simulink model "Tphase"  (R2017a)
settings: Solver=FixedStepDiscrete  StartTime=0.0  StopTime=0.125 - 5e-5  MaxStep=1e-4  RelTol=1e-3
libraries: powerlib x256, auto_lib x2
settings Model: Creator=ioanna  LastModifiedBy=ioanna

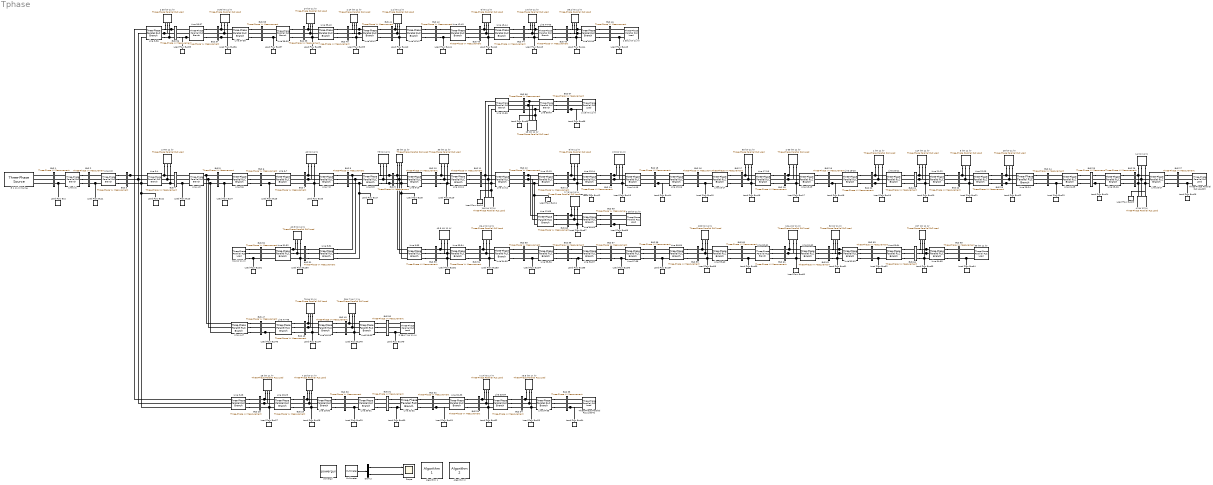
== system Tphase ==
  1 kW 11 kV : powerlib/Elements/Three-Phase Parallel RLC Load  LConnTagsString=A|B|C  Configuration=Y (grounded)  NominalVoltage=11e3  Vabc=[1e3 1e3 1e3]  Vabcp=[1e3 1e3 1e3]  NominalFrequency=50  UnbalancedPower=off  ActivePower=1e3  InductivePower=100  CapacitivePower=0  Pabc=[10e3 9e3 11e3]  QLabc=[100 90 110]  QCabc=[100 90 110]  Pabcp=[10e3 9e3 11e3]  QLabcp=[100 90 110]  QCabcp=[100 90 110]  Measurements=None  LoadType=constant Z
  1.2 kW 11 kV : powerlib/Elements/Three-Phase Parallel RLC Load  LConnTagsString=A|B|C  Configuration=Y (grounded)  NominalVoltage=11e3  Vabc=[1e3 1e3 1e3]  Vabcp=[1e3 1e3 1e3]  NominalFrequency=50  UnbalancedPower=off  ActivePower=1.2e3  InductivePower=100  CapacitivePower=0  Pabc=[10e3 9e3 11e3]  QLabc=[100 90 110]  QCabc=[100 90 110]  Pabcp=[10e3 9e3 11e3]  QLabcp=[100 90 110]  QCabcp=[100 90 110]  Measurements=None  LoadType=constant Z
  100 kW 11 kV : powerlib/Elements/Three-Phase Parallel RLC Load  LConnTagsString=A|B|C  Configuration=Y (grounded)  NominalVoltage=11e3  Vabc=[1e3 1e3 1e3]  Vabcp=[1e3 1e3 1e3]  NominalFrequency=50  UnbalancedPower=off  ActivePower=100e3  InductivePower=100  CapacitivePower=100  Pabc=[10e3 9e3 11e3]  QLabc=[100 90 110]  QCabc=[100 90 110]  Pabcp=[10e3 9e3 11e3]  QLabcp=[100 90 110]  QCabcp=[100 90 110]  Measurements=None  LoadType=constant Z
  114 kW 11 kV : powerlib/Elements/Three-Phase Parallel RLC Load  LConnTagsString=A|B|C  Configuration=Y (grounded)  NominalVoltage=11e3  Vabc=[1e3 1e3 1e3]  Vabcp=[1e3 1e3 1e3]  NominalFrequency=50  UnbalancedPower=off  ActivePower=114e3  InductivePower=100  CapacitivePower=0  Pabc=[10e3 9e3 11e3]  QLabc=[100 90 110]  QCabc=[100 90 110]  Pabcp=[10e3 9e3 11e3]  QLabcp=[100 90 110]  QCabcp=[100 90 110]  Measurements=None  LoadType=constant Z
  1244 kW 11 kV : powerlib/Elements/Three-Phase Parallel RLC Load  LConnTagsString=A|B|C  Configuration=Y (grounded)  NominalVoltage=11e3  Vabc=[1e3 1e3 1e3]  Vabcp=[1e3 1e3 1e3]  NominalFrequency=50  UnbalancedPower=off  ActivePower=1244e3  InductivePower=100  CapacitivePower=100  Pabc=[10e3 9e3 11e3]  QLabc=[100 90 110]  QCabc=[100 90 110]  Pabcp=[10e3 9e3 11e3]  QLabcp=[100 90 110]  QCabcp=[100 90 110]  Measurements=None  LoadType=constant Z
  14 kW 11 kV : powerlib/Elements/Three-Phase Parallel RLC Load  LConnTagsString=A|B|C  Configuration=Y (grounded)  NominalVoltage=11e3  Vabc=[1e3 1e3 1e3]  Vabcp=[1e3 1e3 1e3]  NominalFrequency=50  UnbalancedPower=off  ActivePower=14e3  InductivePower=100  CapacitivePower=0  Pabc=[10e3 9e3 11e3]  QLabc=[100 90 110]  QCabc=[100 90 110]  Pabcp=[10e3 9e3 11e3]  QLabcp=[100 90 110]  QCabcp=[100 90 110]  Measurements=None  LoadType=constant Z
  145 kW 11 kV : powerlib/Elements/Three-Phase Parallel RLC Load  LConnTagsString=A|B|C  Configuration=Y (grounded)  NominalVoltage=11e3  Vabc=[1e3 1e3 1e3]  Vabcp=[1e3 1e3 1e3]  NominalFrequency=50  UnbalancedPower=off  ActivePower=145e3  InductivePower=100  CapacitivePower=0  Pabc=[10e3 9e3 11e3]  QLabc=[100 90 110]  QCabc=[100 90 110]  Pabcp=[10e3 9e3 11e3]  QLabcp=[100 90 110]  QCabcp=[100 90 110]  Measurements=None  LoadType=constant Z
  18 kW 11 kV : powerlib/Elements/Three-Phase Parallel RLC Load  LConnTagsString=A|B|C  Configuration=Y (grounded)  NominalVoltage=11e3  Vabc=[1e3 1e3 1e3]  Vabcp=[1e3 1e3 1e3]  NominalFrequency=50  UnbalancedPower=off  ActivePower=18e3  InductivePower=100  CapacitivePower=0  Pabc=[10e3 9e3 11e3]  QLabc=[100 90 110]  QCabc=[100 90 110]  Pabcp=[10e3 9e3 11e3]  QLabcp=[100 90 110]  QCabcp=[100 90 110]  Measurements=None  LoadType=constant Z
  19.5 kW 11 kV : powerlib/Elements/Three-Phase Parallel RLC Load  LConnTagsString=A|B|C  Configuration=Y (grounded)  NominalVoltage=11e3  Vabc=[1e3 1e3 1e3]  Vabcp=[1e3 1e3 1e3]  NominalFrequency=50  UnbalancedPower=off  ActivePower=19.5e3  InductivePower=100  CapacitivePower=100  Pabc=[10e3 9e3 11e3]  QLabc=[100 90 110]  QCabc=[100 90 110]  Pabcp=[10e3 9e3 11e3]  QLabcp=[100 90 110]  QCabcp=[100 90 110]  Measurements=None  LoadType=constant Z
  2 14 kW 11 kV : powerlib/Elements/Three-Phase Parallel RLC Load  LConnTagsString=A|B|C  Configuration=Y (grounded)  NominalVoltage=11e3  Vabc=[1e3 1e3 1e3]  Vabcp=[1e3 1e3 1e3]  NominalFrequency=50  UnbalancedPower=off  ActivePower=14e3  InductivePower=100  CapacitivePower=100  Pabc=[10e3 9e3 11e3]  QLabc=[100 90 110]  QCabc=[100 90 110]  Pabcp=[10e3 9e3 11e3]  QLabcp=[100 90 110]  QCabcp=[100 90 110]  Measurements=None  LoadType=constant Z
  2 18 kW 11 kV : powerlib/Elements/Three-Phase Parallel RLC Load  LConnTagsString=A|B|C  Configuration=Y (grounded)  NominalVoltage=11e3  Vabc=[1e3 1e3 1e3]  Vabcp=[1e3 1e3 1e3]  NominalFrequency=50  UnbalancedPower=off  ActivePower=18e3  InductivePower=100  CapacitivePower=100  Pabc=[10e3 9e3 11e3]  QLabc=[100 90 110]  QCabc=[100 90 110]  Pabcp=[10e3 9e3 11e3]  QLabcp=[100 90 110]  QCabcp=[100 90 110]  Measurements=None  LoadType=constant Z
  2 24 kW 11 kV : powerlib/Elements/Three-Phase Parallel RLC Load  LConnTagsString=A|B|C  Configuration=Y (grounded)  NominalVoltage=11e3  Vabc=[1e3 1e3 1e3]  Vabcp=[1e3 1e3 1e3]  NominalFrequency=50  UnbalancedPower=off  ActivePower=24e3  InductivePower=100  CapacitivePower=0  Pabc=[10e3 9e3 11e3]  QLabc=[100 90 110]  QCabc=[100 90 110]  Pabcp=[10e3 9e3 11e3]  QLabcp=[100 90 110]  QCabcp=[100 90 110]  Measurements=None  LoadType=constant Z
  2 26 kW 11 kV : powerlib/Elements/Three-Phase Parallel RLC Load  LConnTagsString=A|B|C  Configuration=Y (grounded)  NominalVoltage=11e3  Vabc=[1e3 1e3 1e3]  Vabcp=[1e3 1e3 1e3]  NominalFrequency=50  UnbalancedPower=off  ActivePower=26e3  InductivePower=100  CapacitivePower=100  Pabc=[10e3 9e3 11e3]  QLabc=[100 90 110]  QCabc=[100 90 110]  Pabcp=[10e3 9e3 11e3]  QLabcp=[100 90 110]  QCabcp=[100 90 110]  Measurements=None  LoadType=constant Z
  2 28 kW 11 kV : powerlib/Elements/Three-Phase Parallel RLC Load  LConnTagsString=A|B|C  Configuration=Y (grounded)  NominalVoltage=11e3  Vabc=[1e3 1e3 1e3]  Vabcp=[1e3 1e3 1e3]  NominalFrequency=50  UnbalancedPower=off  ActivePower=28e3  InductivePower=100  CapacitivePower=0  Pabc=[10e3 9e3 11e3]  QLabc=[100 90 110]  QCabc=[100 90 110]  Pabcp=[10e3 9e3 11e3]  QLabcp=[100 90 110]  QCabcp=[100 90 110]  Measurements=None  LoadType=constant Z
  2 30 kW 11 kV : powerlib/Elements/Three-Phase Parallel RLC Load  LConnTagsString=A|B|C  Configuration=Y (grounded)  NominalVoltage=11e3  Vabc=[1e3 1e3 1e3]  Vabcp=[1e3 1e3 1e3]  NominalFrequency=50  UnbalancedPower=off  ActivePower=30e3  InductivePower=100  CapacitivePower=0  Pabc=[10e3 9e3 11e3]  QLabc=[100 90 110]  QCabc=[100 90 110]  Pabcp=[10e3 9e3 11e3]  QLabcp=[100 90 110]  QCabcp=[100 90 110]  Measurements=None  LoadType=constant Z
  2 384.7 kW 11 kV : powerlib/Elements/Three-Phase Parallel RLC Load  LConnTagsString=A|B|C  Configuration=Y (grounded)  NominalVoltage=11e3  Vabc=[1e3 1e3 1e3]  Vabcp=[1e3 1e3 1e3]  NominalFrequency=50  UnbalancedPower=off  ActivePower=384.7e3  InductivePower=100  CapacitivePower=0  Pabc=[10e3 9e3 11e3]  QLabc=[100 90 110]  QCabc=[100 90 110]  Pabcp=[10e3 9e3 11e3]  QLabcp=[100 90 110]  QCabcp=[100 90 110]  Measurements=None  LoadType=constant Z
  2 39.2 kW 11 kV : powerlib/Elements/Three-Phase Parallel RLC Load  LConnTagsString=A|B|C  Configuration=Y (grounded)  NominalVoltage=11e3  Vabc=[1e3 1e3 1e3]  Vabcp=[1e3 1e3 1e3]  NominalFrequency=50  UnbalancedPower=off  ActivePower=39.2e3  InductivePower=100  CapacitivePower=100  Pabc=[10e3 9e3 11e3]  QLabc=[100 90 110]  QCabc=[100 90 110]  Pabcp=[10e3 9e3 11e3]  QLabcp=[100 90 110]  QCabcp=[100 90 110]  Measurements=None  LoadType=constant Z
  2 6 kW 11 kV : powerlib/Elements/Three-Phase Parallel RLC Load  LConnTagsString=A|B|C  Configuration=Y (grounded)  NominalVoltage=11e3  Vabc=[1e3 1e3 1e3]  Vabcp=[1e3 1e3 1e3]  NominalFrequency=50  UnbalancedPower=off  ActivePower=6e3  InductivePower=100  CapacitivePower=100  Pabc=[10e3 9e3 11e3]  QLabc=[100 90 110]  QCabc=[100 90 110]  Pabcp=[10e3 9e3 11e3]  QLabcp=[100 90 110]  QCabcp=[100 90 110]  Measurements=None  LoadType=constant Z
  2 60 kW 11 kV : powerlib/Elements/Three-Phase Parallel RLC Load  LConnTagsString=A|B|C  Configuration=Y (grounded)  NominalVoltage=11e3  Vabc=[1e3 1e3 1e3]  Vabcp=[1e3 1e3 1e3]  NominalFrequency=50  UnbalancedPower=off  ActivePower=60e3  InductivePower=100  CapacitivePower=0  Pabc=[10e3 9e3 11e3]  QLabc=[100 90 110]  QCabc=[100 90 110]  Pabcp=[10e3 9e3 11e3]  QLabcp=[100 90 110]  QCabcp=[100 90 110]  Measurements=None  LoadType=constant Z
  2 8 kW 11 kV : powerlib/Elements/Three-Phase Parallel RLC Load  LConnTagsString=A|B|C  Configuration=Y (grounded)  NominalVoltage=11e3  Vabc=[1e3 1e3 1e3]  Vabcp=[1e3 1e3 1e3]  NominalFrequency=50  UnbalancedPower=off  ActivePower=8e3  InductivePower=100  CapacitivePower=0  Pabc=[10e3 9e3 11e3]  QLabc=[100 90 110]  QCabc=[100 90 110]  Pabcp=[10e3 9e3 11e3]  QLabcp=[100 90 110]  QCabcp=[100 90 110]  Measurements=None  LoadType=constant Z
  2 MW 11 kV : powerlib/Elements/Three-Phase Parallel RLC Load  LConnTagsString=A|B|C  Configuration=Y (grounded)  NominalVoltage=11e3  Vabc=[1e3 1e3 1e3]  Vabcp=[1e3 1e3 1e3]  NominalFrequency=50  UnbalancedPower=off  ActivePower=2e6  InductivePower=100  CapacitivePower=100  Pabc=[10e3 9e3 11e3]  QLabc=[100 90 110]  QCabc=[100 90 110]  Pabcp=[10e3 9e3 11e3]  QLabcp=[100 90 110]  QCabcp=[100 90 110]  Measurements=Branch voltages and currents  LoadType=constant Z
  227 kW 11 kV : powerlib/Elements/Three-Phase Parallel RLC Load  LConnTagsString=A|B|C  Configuration=Y (grounded)  NominalVoltage=11e3  Vabc=[1e3 1e3 1e3]  Vabcp=[1e3 1e3 1e3]  NominalFrequency=50  UnbalancedPower=off  ActivePower=227e3  InductivePower=100  CapacitivePower=100  Pabc=[10e3 9e3 11e3]  QLabc=[100 90 110]  QCabc=[100 90 110]  Pabcp=[10e3 9e3 11e3]  QLabcp=[100 90 110]  QCabcp=[100 90 110]  Measurements=None  LoadType=constant Z
  24 kW 11 kV : powerlib/Elements/Three-Phase Parallel RLC Load  LConnTagsString=A|B|C  Configuration=Y (grounded)  NominalVoltage=11e3  Vabc=[1e3 1e3 1e3]  Vabcp=[1e3 1e3 1e3]  NominalFrequency=50  UnbalancedPower=off  ActivePower=24e3  InductivePower=100  CapacitivePower=0  Pabc=[10e3 9e3 11e3]  QLabc=[100 90 110]  QCabc=[100 90 110]  Pabcp=[10e3 9e3 11e3]  QLabcp=[100 90 110]  QCabcp=[100 90 110]  Measurements=None  LoadType=constant Z
  26 kW 11 kV : powerlib/Elements/Three-Phase Parallel RLC Load  LConnTagsString=A|B|C  Configuration=Y (grounded)  NominalVoltage=11e3  Vabc=[1e3 1e3 1e3]  Vabcp=[1e3 1e3 1e3]  NominalFrequency=50  UnbalancedPower=off  ActivePower=26e3  InductivePower=100  CapacitivePower=100  Pabc=[10e3 9e3 11e3]  QLabc=[100 90 110]  QCabc=[100 90 110]  Pabcp=[10e3 9e3 11e3]  QLabcp=[100 90 110]  QCabcp=[100 90 110]  Measurements=None  LoadType=constant Z
  26.4 kW 11 kV : powerlib/Elements/Three-Phase Parallel RLC Load  LConnTagsString=A|B|C  Configuration=Y (grounded)  NominalVoltage=11e3  Vabc=[1e3 1e3 1e3]  Vabcp=[1e3 1e3 1e3]  NominalFrequency=50  UnbalancedPower=off  ActivePower=26.4e3  InductivePower=100  CapacitivePower=100  Pabc=[10e3 9e3 11e3]  QLabc=[100 90 110]  QCabc=[100 90 110]  Pabcp=[10e3 9e3 11e3]  QLabcp=[100 90 110]  QCabcp=[100 90 110]  Measurements=None  LoadType=constant Z
  28 kW 11 kV : powerlib/Elements/Three-Phase Parallel RLC Load  LConnTagsString=A|B|C  Configuration=Y (grounded)  NominalVoltage=11e3  Vabc=[1e3 1e3 1e3]  Vabcp=[1e3 1e3 1e3]  NominalFrequency=50  UnbalancedPower=off  ActivePower=28e3  InductivePower=100  CapacitivePower=0  Pabc=[10e3 9e3 11e3]  QLabc=[100 90 110]  QCabc=[100 90 110]  Pabcp=[10e3 9e3 11e3]  QLabcp=[100 90 110]  QCabcp=[100 90 110]  Measurements=None  LoadType=constant Z
  3 28 kW 11 kV : powerlib/Elements/Three-Phase Parallel RLC Load  LConnTagsString=A|B|C  Configuration=Y (grounded)  NominalVoltage=11e3  Vabc=[1e3 1e3 1e3]  Vabcp=[1e3 1e3 1e3]  NominalFrequency=50  UnbalancedPower=off  ActivePower=28e3  InductivePower=100  CapacitivePower=0  Pabc=[10e3 9e3 11e3]  QLabc=[100 90 110]  QCabc=[100 90 110]  Pabcp=[10e3 9e3 11e3]  QLabcp=[100 90 110]  QCabcp=[100 90 110]  Measurements=None  LoadType=constant Z
  3 30 kW 11 kV : powerlib/Elements/Three-Phase Parallel RLC Load  LConnTagsString=A|B|C  Configuration=Y (grounded)  NominalVoltage=11e3  Vabc=[1e3 1e3 1e3]  Vabcp=[1e3 1e3 1e3]  NominalFrequency=50  UnbalancedPower=off  ActivePower=30e3  InductivePower=100  CapacitivePower=0  Pabc=[10e3 9e3 11e3]  QLabc=[100 90 110]  QCabc=[100 90 110]  Pabcp=[10e3 9e3 11e3]  QLabcp=[100 90 110]  QCabcp=[100 90 110]  Measurements=None  LoadType=constant Z
  3.6 kW 11 kV : powerlib/Elements/Three-Phase Parallel RLC Load  LConnTagsString=A|B|C  Configuration=Y (grounded)  NominalVoltage=11e3  Vabc=[1e3 1e3 1e3]  Vabcp=[1e3 1e3 1e3]  NominalFrequency=50  UnbalancedPower=off  ActivePower=3.6e3  InductivePower=100  CapacitivePower=100  Pabc=[10e3 9e3 11e3]  QLabc=[100 90 110]  QCabc=[100 90 110]  Pabcp=[10e3 9e3 11e3]  QLabcp=[100 90 110]  QCabcp=[100 90 110]  Measurements=None  LoadType=constant Z
  30 kW 11 kV : powerlib/Elements/Three-Phase Parallel RLC Load  LConnTagsString=A|B|C  Configuration=Y (grounded)  NominalVoltage=11e3  Vabc=[1e3 1e3 1e3]  Vabcp=[1e3 1e3 1e3]  NominalFrequency=50  UnbalancedPower=off  ActivePower=30e3  InductivePower=100  CapacitivePower=1000  Pabc=[10e3 9e3 11e3]  QLabc=[100 90 110]  QCabc=[100 90 110]  Pabcp=[10e3 9e3 11e3]  QLabcp=[100 90 110]  QCabcp=[100 90 110]  Measurements=None  LoadType=constant Z
  30 kW 11 kV : powerlib/Elements/Three-Phase Parallel RLC Load  LConnTagsString=A|B|C  Configuration=Y (grounded)  NominalVoltage=11e3  Vabc=[1e3 1e3 1e3]  Vabcp=[1e3 1e3 1e3]  NominalFrequency=50  UnbalancedPower=off  ActivePower=30e3  InductivePower=100  CapacitivePower=0  Pabc=[10e3 9e3 11e3]  QLabc=[100 90 110]  QCabc=[100 90 110]  Pabcp=[10e3 9e3 11e3]  QLabcp=[100 90 110]  QCabcp=[100 90 110]  Measurements=None  LoadType=constant Z
  32 kW 11 kV : powerlib/Elements/Three-Phase Parallel RLC Load  LConnTagsString=A|B|C  Configuration=Y (grounded)  NominalVoltage=11e3  Vabc=[1e3 1e3 1e3]  Vabcp=[1e3 1e3 1e3]  NominalFrequency=50  UnbalancedPower=off  ActivePower=32e3  InductivePower=100  CapacitivePower=100  Pabc=[10e3 9e3 11e3]  QLabc=[100 90 110]  QCabc=[100 90 110]  Pabcp=[10e3 9e3 11e3]  QLabcp=[100 90 110]  QCabcp=[100 90 110]  Measurements=None  LoadType=constant Z
  384.7 kW 11 kV : powerlib/Elements/Three-Phase Parallel RLC Load  LConnTagsString=A|B|C  Configuration=Y (grounded)  NominalVoltage=11e3  Vabc=[1e3 1e3 1e3]  Vabcp=[1e3 1e3 1e3]  NominalFrequency=50  UnbalancedPower=off  ActivePower=384.7e3  InductivePower=100  CapacitivePower=0  Pabc=[10e3 9e3 11e3]  QLabc=[100 90 110]  QCabc=[100 90 110]  Pabcp=[10e3 9e3 11e3]  QLabcp=[100 90 110]  QCabcp=[100 90 110]  Measurements=None  LoadType=constant Z
  39.2 kW 11 kV : powerlib/Elements/Three-Phase Parallel RLC Load  LConnTagsString=A|B|C  Configuration=Y (grounded)  NominalVoltage=11e3  Vabc=[1e3 1e3 1e3]  Vabcp=[1e3 1e3 1e3]  NominalFrequency=50  UnbalancedPower=off  ActivePower=39.2e3  InductivePower=100  CapacitivePower=100  Pabc=[10e3 9e3 11e3]  QLabc=[100 90 110]  QCabc=[100 90 110]  Pabcp=[10e3 9e3 11e3]  QLabcp=[100 90 110]  QCabcp=[100 90 110]  Measurements=None  LoadType=constant Z
  4 MW 11 kV : powerlib/Elements/Three-Phase Parallel RLC Load  LConnTagsString=A|B|C  Configuration=Y (grounded)  NominalVoltage=11e3  Vabc=[1e3 1e3 1e3]  Vabcp=[1e3 1e3 1e3]  NominalFrequency=50  UnbalancedPower=off  ActivePower=4e6  InductivePower=100  CapacitivePower=100  Pabc=[10e3 9e3 11e3]  QLabc=[100 90 110]  QCabc=[100 90 110]  Pabcp=[10e3 9e3 11e3]  QLabcp=[100 90 110]  QCabcp=[100 90 110]  Measurements=None  LoadType=constant Z
  40 kW 11 kV : powerlib/Elements/Three-Phase Parallel RLC Load  LConnTagsString=A|B|C  Configuration=Y (grounded)  NominalVoltage=11e3  Vabc=[1e3 1e3 1e3]  Vabcp=[1e3 1e3 1e3]  NominalFrequency=50  UnbalancedPower=off  ActivePower=40e3  InductivePower=0  CapacitivePower=100  Pabc=[10e3 9e3 11e3]  QLabc=[100 90 110]  QCabc=[100 90 110]  Pabcp=[10e3 9e3 11e3]  QLabcp=[100 90 110]  QCabcp=[100 90 110]  Measurements=None  LoadType=constant Z
  40.5 kW 11 kV : powerlib/Elements/Three-Phase Parallel RLC Load  LConnTagsString=A|B|C  Configuration=Y (grounded)  NominalVoltage=11e3  Vabc=[1e3 1e3 1e3]  Vabcp=[1e3 1e3 1e3]  NominalFrequency=50  UnbalancedPower=off  ActivePower=40.5e3  InductivePower=100  CapacitivePower=0  Pabc=[10e3 9e3 11e3]  QLabc=[100 90 110]  QCabc=[100 90 110]  Pabcp=[10e3 9e3 11e3]  QLabcp=[100 90 110]  QCabcp=[100 90 110]  Measurements=None  LoadType=constant Z
  43.5 kW 11 kV : powerlib/Elements/Three-Phase Parallel RLC Load  LConnTagsString=A|B|C  Configuration=Y (grounded)  NominalVoltage=11e3  Vabc=[1e3 1e3 1e3]  Vabcp=[1e3 1e3 1e3]  NominalFrequency=50  UnbalancedPower=off  ActivePower=43.5e3  InductivePower=100  CapacitivePower=100  Pabc=[10e3 9e3 11e3]  QLabc=[100 90 110]  QCabc=[100 90 110]  Pabcp=[10e3 9e3 11e3]  QLabcp=[100 90 110]  QCabcp=[100 90 110]  Measurements=None  LoadType=constant Z
  5 kW 11 kV : powerlib/Elements/Three-Phase Parallel RLC Load  LConnTagsString=A|B|C  Configuration=Y (grounded)  NominalVoltage=11e3  Vabc=[1e3 1e3 1e3]  Vabcp=[1e3 1e3 1e3]  NominalFrequency=50  UnbalancedPower=off  ActivePower=5e3  InductivePower=100  CapacitivePower=0  Pabc=[10e3 9e3 11e3]  QLabc=[100 90 110]  QCabc=[100 90 110]  Pabcp=[10e3 9e3 11e3]  QLabcp=[100 90 110]  QCabcp=[100 90 110]  Measurements=None  LoadType=constant Z
  59 kW 11 kV : powerlib/Elements/Three-Phase Parallel RLC Load  LConnTagsString=A|B|C  Configuration=Y (grounded)  NominalVoltage=11e3  Vabc=[1e3 1e3 1e3]  Vabcp=[1e3 1e3 1e3]  NominalFrequency=50  UnbalancedPower=off  ActivePower=59e3  InductivePower=100  CapacitivePower=100  Pabc=[10e3 9e3 11e3]  QLabc=[100 90 110]  QCabc=[100 90 110]  Pabcp=[10e3 9e3 11e3]  QLabcp=[100 90 110]  QCabcp=[100 90 110]  Measurements=None  LoadType=constant Z
  6 kW 11 kV : powerlib/Elements/Three-Phase Parallel RLC Load  LConnTagsString=A|B|C  Configuration=Y (grounded)  NominalVoltage=11e3  Vabc=[1e3 1e3 1e3]  Vabcp=[1e3 1e3 1e3]  NominalFrequency=50  UnbalancedPower=off  ActivePower=6e3  InductivePower=100  CapacitivePower=100  Pabc=[10e3 9e3 11e3]  QLabc=[100 90 110]  QCabc=[100 90 110]  Pabcp=[10e3 9e3 11e3]  QLabcp=[100 90 110]  QCabcp=[100 90 110]  Measurements=None  LoadType=constant Z
  60 kW 11 kV : powerlib/Elements/Three-Phase Parallel RLC Load  LConnTagsString=A|B|C  Configuration=Y (grounded)  NominalVoltage=11e3  Vabc=[1e3 1e3 1e3]  Vabcp=[1e3 1e3 1e3]  NominalFrequency=50  UnbalancedPower=off  ActivePower=60e3  InductivePower=100  CapacitivePower=0  Pabc=[10e3 9e3 11e3]  QLabc=[100 90 110]  QCabc=[100 90 110]  Pabcp=[10e3 9e3 11e3]  QLabcp=[100 90 110]  QCabcp=[100 90 110]  Measurements=None  LoadType=constant Z
  75 kW 11 kV : powerlib/Elements/Three-Phase Parallel RLC Load  LConnTagsString=A|B|C  Configuration=Y (grounded)  NominalVoltage=11e3  Vabc=[1e3 1e3 1e3]  Vabcp=[1e3 1e3 1e3]  NominalFrequency=50  UnbalancedPower=off  ActivePower=75e3  InductivePower=100  CapacitivePower=0  Pabc=[10e3 9e3 11e3]  QLabc=[100 90 110]  QCabc=[100 90 110]  Pabcp=[10e3 9e3 11e3]  QLabcp=[100 90 110]  QCabcp=[100 90 110]  Measurements=None  LoadType=constant Z
  79 kW 11 kV : powerlib/Elements/Three-Phase Parallel RLC Load  LConnTagsString=A|B|C  Configuration=Y (grounded)  NominalVoltage=11e3  Vabc=[1e3 1e3 1e3]  Vabcp=[1e3 1e3 1e3]  NominalFrequency=50  UnbalancedPower=off  ActivePower=79e3  InductivePower=100  CapacitivePower=0  Pabc=[10e3 9e3 11e3]  QLabc=[100 90 110]  QCabc=[100 90 110]  Pabcp=[10e3 9e3 11e3]  QLabcp=[100 90 110]  QCabcp=[100 90 110]  Measurements=None  LoadType=constant Z
  8 kW 11 kV : powerlib/Elements/Three-Phase Parallel RLC Load  LConnTagsString=A|B|C  Configuration=Y (grounded)  NominalVoltage=11e3  Vabc=[1e3 1e3 1e3]  Vabcp=[1e3 1e3 1e3]  NominalFrequency=50  UnbalancedPower=off  ActivePower=8e3  InductivePower=100  CapacitivePower=0  Pabc=[10e3 9e3 11e3]  QLabc=[100 90 110]  QCabc=[100 90 110]  Pabcp=[10e3 9e3 11e3]  QLabcp=[100 90 110]  QCabcp=[100 90 110]  Measurements=None  LoadType=constant Z
  Algorithm 1 : auto_lib/Algorithm 1  SystemSampleTime=-1
  Algorithm 2 : auto_lib/Algorithm 2  SystemSampleTime=-1
  BUS {1..69} (69 alike) : powerlib/Measurements/Three-Phase V-I Measurement  VoltageMeasurement=no  SetLabelV=off  LabelV=Vabc  Vpu=off  VpuLL=off  CurrentMeasurement=no  SetLabelI=off  LabelI=Iabc  Ipu=off  Pbase=100e6  Vbase=500e3  OutputType=Complex  PhasorSimulation=off  PSBequivalent=0
  Demux : Demux  Outputs=2
  G 1 11 kV Swing : powerlib/Electrical Sources/Three-Phase Source  InternalConnection=Yg  VoltagePhases=off  Voltage=11e3  PhaseAngle=0  Voltage_phases=[25e3 25e3 25e3]/sqrt(3)  PhaseAngles_phases=[0 -120 +120]  Frequency=50  NonIdealSource=on  SpecifyImpedance=off  Resistance=0.8929  Inductance=16.58e-3  ShortCircuitLevel=100e6  BaseVoltage=25e3  XRratio=7  BusType=swing  Pref=10e3  Qref=0  Prefabc=[10e3, 10e3, 10e3]  Qrefabc=[0, 0, 0]  Qmin=-inf  Qmax=inf
  Line 1-2 : powerlib/Elements/Three-Phase Parallel RLC Branch  LConnTagsString=A|B|C  RConnTagsString=A|B|C  BranchType=RL  Resistance=0.0005  Inductance=0.0012  Capacitance=1e-6  Measurements=None
      settings: SourceProductName=Simscape Power Systems  SourceProductBaseCode=PS
  Line 10-11 : powerlib/Elements/Three-Phase Parallel RLC Branch  LConnTagsString=A|B|C  RConnTagsString=A|B|C  BranchType=RL  Resistance=0.1872  Inductance=0.0619  Capacitance=1e-6  Measurements=None
      settings: SourceProductName=Simscape Power Systems  SourceProductBaseCode=PS
  Line 11-12 : powerlib/Elements/Three-Phase Parallel RLC Branch  LConnTagsString=A|B|C  RConnTagsString=A|B|C  BranchType=RL  Resistance=0.7114  Inductance=0.2351  Capacitance=1e-6  Measurements=None
      settings: SourceProductName=Simscape Power Systems  SourceProductBaseCode=PS
  Line 11-66 : powerlib/Elements/Three-Phase Parallel RLC Branch  LConnTagsString=A|B|C  RConnTagsString=A|B|C  BranchType=RL  Resistance=0.2012  Inductance=0.0611  Capacitance=1e-6  Measurements=None
      settings: SourceProductName=Simscape Power Systems  SourceProductBaseCode=PS
  Line 12-13 : powerlib/Elements/Three-Phase Parallel RLC Branch  LConnTagsString=A|B|C  RConnTagsString=A|B|C  BranchType=RL  Resistance=1.03  Inductance=0.34  Capacitance=1e-6  Measurements=None
      settings: SourceProductName=Simscape Power Systems  SourceProductBaseCode=PS
  Line 12-68 : powerlib/Elements/Three-Phase Parallel RLC Branch  LConnTagsString=A|B|C  RConnTagsString=A|B|C  BranchType=RL  Resistance=0.7394  Inductance=0.2444  Capacitance=1e-6  Measurements=None
      settings: SourceProductName=Simscape Power Systems  SourceProductBaseCode=PS
  Line 13-14 : powerlib/Elements/Three-Phase Parallel RLC Branch  LConnTagsString=A|B|C  RConnTagsString=A|B|C  BranchType=RL  Resistance=1.044  Inductance=0.345  Capacitance=1e-6  Measurements=None
      settings: SourceProductName=Simscape Power Systems  SourceProductBaseCode=PS
  Line 14-15 : powerlib/Elements/Three-Phase Parallel RLC Branch  LConnTagsString=A|B|C  RConnTagsString=A|B|C  BranchType=RL  Resistance=1.058  Inductance=0.3496  Capacitance=1e-6  Measurements=None
      settings: SourceProductName=Simscape Power Systems  SourceProductBaseCode=PS
  Line 15-16 : powerlib/Elements/Three-Phase Parallel RLC Branch  LConnTagsString=A|B|C  RConnTagsString=A|B|C  BranchType=RL  Resistance=0.1966  Inductance=0.065  Capacitance=1e-6  Measurements=None
      settings: SourceProductName=Simscape Power Systems  SourceProductBaseCode=PS
  Line 16-17 : powerlib/Elements/Three-Phase Parallel RLC Branch  LConnTagsString=A|B|C  RConnTagsString=A|B|C  BranchType=RL  Resistance=0.3744  Inductance=0.1238  Capacitance=1e-6  Measurements=None
      settings: SourceProductName=Simscape Power Systems  SourceProductBaseCode=PS
  Line 17-18 : powerlib/Elements/Three-Phase Parallel RLC Branch  LConnTagsString=A|B|C  RConnTagsString=A|B|C  BranchType=RL  Resistance=0.0047  Inductance=0.0016  Capacitance=1e-6  Measurements=None
      settings: SourceProductName=Simscape Power Systems  SourceProductBaseCode=PS
  Line 18-19 : powerlib/Elements/Three-Phase Parallel RLC Branch  LConnTagsString=A|B|C  RConnTagsString=A|B|C  BranchType=RL  Resistance=0.3276  Inductance=0.1083  Capacitance=1e-6  Measurements=None
      settings: SourceProductName=Simscape Power Systems  SourceProductBaseCode=PS
  Line 19-20 : powerlib/Elements/Three-Phase Parallel RLC Branch  LConnTagsString=A|B|C  RConnTagsString=A|B|C  BranchType=RL  Resistance=0.2106  Inductance=0.069  Capacitance=1e-6  Measurements=None
      settings: SourceProductName=Simscape Power Systems  SourceProductBaseCode=PS
  Line 2-3 : powerlib/Elements/Three-Phase Parallel RLC Branch  LConnTagsString=A|B|C  RConnTagsString=A|B|C  BranchType=RL  Resistance=0.0005  Inductance=0.0012  Capacitance=1e-6  Measurements=None
      settings: SourceProductName=Simscape Power Systems  SourceProductBaseCode=PS
  Line 20-21 : powerlib/Elements/Three-Phase Parallel RLC Branch  LConnTagsString=A|B|C  RConnTagsString=A|B|C  BranchType=RL  Resistance=0.3416  Inductance=0.1129  Capacitance=1e-6  Measurements=None
      settings: SourceProductName=Simscape Power Systems  SourceProductBaseCode=PS
  Line 21-22 : powerlib/Elements/Three-Phase Parallel RLC Branch  LConnTagsString=A|B|C  RConnTagsString=A|B|C  BranchType=RL  Resistance=0.014  Inductance=0.0046  Capacitance=1e-6  Measurements=None
      settings: SourceProductName=Simscape Power Systems  SourceProductBaseCode=PS
  Line 22-23 : powerlib/Elements/Three-Phase Parallel RLC Branch  LConnTagsString=A|B|C  RConnTagsString=A|B|C  BranchType=RL  Resistance=0.1591  Inductance=0.0526  Capacitance=1e-6  Measurements=None
      settings: SourceProductName=Simscape Power Systems  SourceProductBaseCode=PS
  Line 23-24 : powerlib/Elements/Three-Phase Parallel RLC Branch  LConnTagsString=A|B|C  RConnTagsString=A|B|C  BranchType=RL  Resistance=0.3469  Inductance=0.1145  Capacitance=1e-6  Measurements=None
      settings: SourceProductName=Simscape Power Systems  SourceProductBaseCode=PS
  Line 24-25 : powerlib/Elements/Three-Phase Parallel RLC Branch  LConnTagsString=A|B|C  RConnTagsString=A|B|C  BranchType=RL  Resistance=0.7488  Inductance=0.2475  Capacitance=1e-6  Measurements=None
      settings: SourceProductName=Simscape Power Systems  SourceProductBaseCode=PS
  Line 25-26 : powerlib/Elements/Three-Phase Parallel RLC Branch  LConnTagsString=A|B|C  RConnTagsString=A|B|C  BranchType=RL  Resistance=0.3089  Inductance=0.1021  Capacitance=1e-6  Measurements=None
      settings: SourceProductName=Simscape Power Systems  SourceProductBaseCode=PS
  Line 26-27 : powerlib/Elements/Three-Phase Parallel RLC Branch  LConnTagsString=A|B|C  RConnTagsString=A|B|C  BranchType=RL  Resistance=0.1732  Inductance=0.0572  Capacitance=1e-6  Measurements=None
      settings: SourceProductName=Simscape Power Systems  SourceProductBaseCode=PS
  Line 28-29 : powerlib/Elements/Three-Phase Parallel RLC Branch  LConnTagsString=A|B|C  RConnTagsString=A|B|C  BranchType=RL  Resistance=0.064  Inductance=0.1565  Capacitance=1e-6  Measurements=None
      settings: SourceProductName=Simscape Power Systems  SourceProductBaseCode=PS
  Line 29-30 : powerlib/Elements/Three-Phase Parallel RLC Branch  LConnTagsString=A|B|C  RConnTagsString=A|B|C  BranchType=RL  Resistance=0.3978  Inductance=0.1315  Capacitance=1e-6  Measurements=None
      settings: SourceProductName=Simscape Power Systems  SourceProductBaseCode=PS
  Line 3-28 : powerlib/Elements/Three-Phase Parallel RLC Branch  LConnTagsString=A|B|C  RConnTagsString=A|B|C  BranchType=RL  Resistance=0.0005  Inductance=0.0036  Capacitance=1e-6  Measurements=None
      settings: SourceProductName=Simscape Power Systems  SourceProductBaseCode=PS
  Line 3-36 : powerlib/Elements/Three-Phase Parallel RLC Branch  LConnTagsString=A|B|C  RConnTagsString=A|B|C  BranchType=RL  Resistance=0.0005  Inductance=0.0036  Capacitance=1e-6  Measurements=None
      settings: SourceProductName=Simscape Power Systems  SourceProductBaseCode=PS
  Line 3-4 : powerlib/Elements/Three-Phase Parallel RLC Branch  LConnTagsString=A|B|C  RConnTagsString=A|B|C  BranchType=RL  Resistance=0.0005  Inductance=0.0036  Capacitance=1e-6  Measurements=None
      settings: SourceProductName=Simscape Power Systems  SourceProductBaseCode=PS
  Line 30-31 : powerlib/Elements/Three-Phase Parallel RLC Branch  LConnTagsString=A|B|C  RConnTagsString=A|B|C  BranchType=RL  Resistance=0.0702  Inductance=0.0232  Capacitance=1e-6  Measurements=None
      settings: SourceProductName=Simscape Power Systems  SourceProductBaseCode=PS
  Line 31-32 : powerlib/Elements/Three-Phase Parallel RLC Branch  LConnTagsString=A|B|C  RConnTagsString=A|B|C  BranchType=RL  Resistance=0.351  Inductance=0.116  Capacitance=1e-6  Measurements=None
      settings: SourceProductName=Simscape Power Systems  SourceProductBaseCode=PS
  Line 32-33 : powerlib/Elements/Three-Phase Parallel RLC Branch  LConnTagsString=A|B|C  RConnTagsString=A|B|C  BranchType=RL  Resistance=0.839  Inductance=0.2816  Capacitance=1e-6  Measurements=None
      settings: SourceProductName=Simscape Power Systems  SourceProductBaseCode=PS
  Line 33-34 : powerlib/Elements/Three-Phase Parallel RLC Branch  LConnTagsString=A|B|C  RConnTagsString=A|B|C  BranchType=RL  Resistance=1.708  Inductance=0.5646  Capacitance=1e-6  Measurements=None
      settings: SourceProductName=Simscape Power Systems  SourceProductBaseCode=PS
  Line 34-35 : powerlib/Elements/Three-Phase Parallel RLC Branch  LConnTagsString=A|B|C  RConnTagsString=A|B|C  BranchType=RL  Resistance=1.474  Inductance=0.4873  Capacitance=1e-6  Measurements=None
      settings: SourceProductName=Simscape Power Systems  SourceProductBaseCode=PS
  Line 36-37 : powerlib/Elements/Three-Phase Parallel RLC Branch  LConnTagsString=A|B|C  RConnTagsString=A|B|C  BranchType=RL  Resistance=0.064  Inductance=0.1565  Capacitance=1e-6  Measurements=None
      settings: SourceProductName=Simscape Power Systems  SourceProductBaseCode=PS
  Line 37-38 : powerlib/Elements/Three-Phase Parallel RLC Branch  LConnTagsString=A|B|C  RConnTagsString=A|B|C  BranchType=RL  Resistance=0.1053  Inductance=0.123  Capacitance=1e-6  Measurements=None
      settings: SourceProductName=Simscape Power Systems  SourceProductBaseCode=PS
  Line 38-39 : powerlib/Elements/Three-Phase Parallel RLC Branch  LConnTagsString=A|B|C  RConnTagsString=A|B|C  BranchType=RL  Resistance=0.0304  Inductance=0.0355  Capacitance=1e-6  Measurements=None
      settings: SourceProductName=Simscape Power Systems  SourceProductBaseCode=PS
  Line 39-40 : powerlib/Elements/Three-Phase Parallel RLC Branch  LConnTagsString=A|B|C  RConnTagsString=A|B|C  BranchType=RL  Resistance=0.0018  Inductance=0.0021  Capacitance=1e-6  Measurements=None
      settings: SourceProductName=Simscape Power Systems  SourceProductBaseCode=PS
  Line 4-47 : powerlib/Elements/Three-Phase Parallel RLC Branch  LConnTagsString=A|B|C  RConnTagsString=A|B|C  BranchType=RL  Resistance=0.0034  Inductance=0.0084  Capacitance=1e-6  Measurements=None
      settings: SourceProductName=Simscape Power Systems  SourceProductBaseCode=PS
  Line 4-5 : powerlib/Elements/Three-Phase Parallel RLC Branch  LConnTagsString=A|B|C  RConnTagsString=A|B|C  BranchType=RL  Resistance=0.0251  Inductance=0.0294  Capacitance=1e-6  Measurements=None
      settings: SourceProductName=Simscape Power Systems  SourceProductBaseCode=PS
  Line 40-41 : powerlib/Elements/Three-Phase Parallel RLC Branch  LConnTagsString=A|B|C  RConnTagsString=A|B|C  BranchType=RL  Resistance=0.7283  Inductance=0.8509  Capacitance=1e-6  Measurements=None
      settings: SourceProductName=Simscape Power Systems  SourceProductBaseCode=PS
  Line 41-42 : powerlib/Elements/Three-Phase Parallel RLC Branch  LConnTagsString=A|B|C  RConnTagsString=A|B|C  BranchType=RL  Resistance=0.31  Inductance=0.3623  Capacitance=1e-6  Measurements=None
      settings: SourceProductName=Simscape Power Systems  SourceProductBaseCode=PS
  Line 42-43 : powerlib/Elements/Three-Phase Parallel RLC Branch  LConnTagsString=A|B|C  RConnTagsString=A|B|C  BranchType=RL  Resistance=0.041  Inductance=0.0478  Capacitance=1e-6  Measurements=None
      settings: SourceProductName=Simscape Power Systems  SourceProductBaseCode=PS
  Line 43-44 : powerlib/Elements/Three-Phase Parallel RLC Branch  LConnTagsString=A|B|C  RConnTagsString=A|B|C  BranchType=RL  Resistance=0.0092  Inductance=0.0116  Capacitance=1e-6  Measurements=None
      settings: SourceProductName=Simscape Power Systems  SourceProductBaseCode=PS
  Line 44-45 : powerlib/Elements/Three-Phase Parallel RLC Branch  LConnTagsString=A|B|C  RConnTagsString=A|B|C  BranchType=RL  Resistance=0.1089  Inductance=0.1373  Capacitance=1e-6  Measurements=None
      settings: SourceProductName=Simscape Power Systems  SourceProductBaseCode=PS
  Line 45-46 : powerlib/Elements/Three-Phase Parallel RLC Branch  LConnTagsString=A|B|C  RConnTagsString=A|B|C  BranchType=RL  Resistance=0.0009  Inductance=0.0012  Capacitance=1e-6  Measurements=None
      settings: SourceProductName=Simscape Power Systems  SourceProductBaseCode=PS
  Line 47-48 : powerlib/Elements/Three-Phase Parallel RLC Branch  LConnTagsString=A|B|C  RConnTagsString=A|B|C  BranchType=RL  Resistance=0.0851  Inductance=0.2083  Capacitance=1e-6  Measurements=None
      settings: SourceProductName=Simscape Power Systems  SourceProductBaseCode=PS
  Line 48-49 : powerlib/Elements/Three-Phase Parallel RLC Branch  LConnTagsString=A|B|C  RConnTagsString=A|B|C  BranchType=RL  Resistance=0.2898  Inductance=0.7091  Capacitance=1e-6  Measurements=None
      settings: SourceProductName=Simscape Power Systems  SourceProductBaseCode=PS
  Line 49-50 : powerlib/Elements/Three-Phase Parallel RLC Branch  LConnTagsString=A|B|C  RConnTagsString=A|B|C  BranchType=RL  Resistance=0.0822  Inductance=0.2011  Capacitance=1e-6  Measurements=None
      settings: SourceProductName=Simscape Power Systems  SourceProductBaseCode=PS
  Line 5-6 : powerlib/Elements/Three-Phase Parallel RLC Branch  LConnTagsString=A|B|C  RConnTagsString=A|B|C  BranchType=RL  Resistance=0.366  Inductance=0.1864  Capacitance=1e-6  Measurements=None
      settings: SourceProductName=Simscape Power Systems  SourceProductBaseCode=PS
  Line 51-52 : powerlib/Elements/Three-Phase Parallel RLC Branch  LConnTagsString=A|B|C  RConnTagsString=A|B|C  BranchType=RL  Resistance=0.3319  Inductance=0.1114  Capacitance=1e-6  Measurements=None
      settings: SourceProductName=Simscape Power Systems  SourceProductBaseCode=PS
  Line 53-54 : powerlib/Elements/Three-Phase Parallel RLC Branch  LConnTagsString=A|B|C  RConnTagsString=A|B|C  BranchType=RL  Resistance=0.203  Inductance=0.1034  Capacitance=1e-6  Measurements=None
      settings: SourceProductName=Simscape Power Systems  SourceProductBaseCode=PS
  Line 54-55 : powerlib/Elements/Three-Phase Parallel RLC Branch  LConnTagsString=A|B|C  RConnTagsString=A|B|C  BranchType=RL  Resistance=0.2842  Inductance=0.1447  Capacitance=1e-6  Measurements=None
      settings: SourceProductName=Simscape Power Systems  SourceProductBaseCode=PS
  Line 55-56 : powerlib/Elements/Three-Phase Parallel RLC Branch  LConnTagsString=A|B|C  RConnTagsString=A|B|C  BranchType=RL  Resistance=0.2813  Inductance=0.1443  Capacitance=1e-6  Measurements=None
      settings: SourceProductName=Simscape Power Systems  SourceProductBaseCode=PS
  Line 56-57 : powerlib/Elements/Three-Phase Parallel RLC Branch  LConnTagsString=A|B|C  RConnTagsString=A|B|C  BranchType=RL  Resistance=1.59  Inductance=0.5337  Capacitance=1e-6  Measurements=None
      settings: SourceProductName=Simscape Power Systems  SourceProductBaseCode=PS
  Line 57-58 : powerlib/Elements/Three-Phase Parallel RLC Branch  LConnTagsString=A|B|C  RConnTagsString=A|B|C  BranchType=RL  Resistance=0.7837  Inductance=0.263  Capacitance=1e-6  Measurements=None
      settings: SourceProductName=Simscape Power Systems  SourceProductBaseCode=PS
  Line 58-59 : powerlib/Elements/Three-Phase Parallel RLC Branch  LConnTagsString=A|B|C  RConnTagsString=A|B|C  BranchType=RL  Resistance=0.3042  Inductance=0.1006  Capacitance=1e-6  Measurements=None
      settings: SourceProductName=Simscape Power Systems  SourceProductBaseCode=PS
  Line 59-60 : powerlib/Elements/Three-Phase Parallel RLC Branch  LConnTagsString=A|B|C  RConnTagsString=A|B|C  BranchType=RL  Resistance=0.3861  Inductance=0.1172  Capacitance=1e-6  Measurements=None
      settings: SourceProductName=Simscape Power Systems  SourceProductBaseCode=PS
  Line 6-7 : powerlib/Elements/Three-Phase Parallel RLC Branch  LConnTagsString=A|B|C  RConnTagsString=A|B|C  BranchType=RL  Resistance=0.3811  Inductance=0.1941  Capacitance=1e-6  Measurements=None
      settings: SourceProductName=Simscape Power Systems  SourceProductBaseCode=PS
  Line 60-61 : powerlib/Elements/Three-Phase Parallel RLC Branch  LConnTagsString=A|B|C  RConnTagsString=A|B|C  BranchType=RL  Resistance=0.5075  Inductance=0.2585  Capacitance=1e-6  Measurements=None
      settings: SourceProductName=Simscape Power Systems  SourceProductBaseCode=PS
  Line 61-62 : powerlib/Elements/Three-Phase Parallel RLC Branch  LConnTagsString=A|B|C  RConnTagsString=A|B|C  BranchType=RL  Resistance=0.0974  Inductance=0.0496  Capacitance=1e-6  Measurements=None
      settings: SourceProductName=Simscape Power Systems  SourceProductBaseCode=PS
  Line 62-63 : powerlib/Elements/Three-Phase Parallel RLC Branch  LConnTagsString=A|B|C  RConnTagsString=A|B|C  BranchType=RL  Resistance=0.145  Inductance=0.0738  Capacitance=1e-6  Measurements=None
      settings: SourceProductName=Simscape Power Systems  SourceProductBaseCode=PS
  Line 63-64 : powerlib/Elements/Three-Phase Parallel RLC Branch  LConnTagsString=A|B|C  RConnTagsString=A|B|C  BranchType=RL  Resistance=0.7105  Inductance=0.3619  Capacitance=1e-6  Measurements=None
      settings: SourceProductName=Simscape Power Systems  SourceProductBaseCode=PS
  Line 64-65 : powerlib/Elements/Three-Phase Parallel RLC Branch  LConnTagsString=A|B|C  RConnTagsString=A|B|C  BranchType=RL  Resistance=1.041  Inductance=0.5302  Capacitance=1e-6  Measurements=None
      settings: SourceProductName=Simscape Power Systems  SourceProductBaseCode=PS
  Line 66-67 : powerlib/Elements/Three-Phase Parallel RLC Branch  LConnTagsString=A|B|C  RConnTagsString=A|B|C  BranchType=RL  Resistance=0.0047  Inductance=0.0014  Capacitance=1e-6  Measurements=None
      settings: SourceProductName=Simscape Power Systems  SourceProductBaseCode=PS
  Line 68-69 : powerlib/Elements/Three-Phase Parallel RLC Branch  LConnTagsString=A|B|C  RConnTagsString=A|B|C  BranchType=RL  Resistance=0.0047  Inductance=0.0016  Capacitance=1e-6  Measurements=None
      settings: SourceProductName=Simscape Power Systems  SourceProductBaseCode=PS
  Line 7-8 : powerlib/Elements/Three-Phase Parallel RLC Branch  LConnTagsString=A|B|C  RConnTagsString=A|B|C  BranchType=RL  Resistance=0.0922  Inductance=0.047  Capacitance=1e-6  Measurements=None
      settings: SourceProductName=Simscape Power Systems  SourceProductBaseCode=PS
  Line 8-51 : powerlib/Elements/Three-Phase Parallel RLC Branch  LConnTagsString=A|B|C  RConnTagsString=A|B|C  BranchType=RL  Resistance=0.0928  Inductance=0.0473  Capacitance=1e-6  Measurements=None
      settings: SourceProductName=Simscape Power Systems  SourceProductBaseCode=PS
  Line 8-9 : powerlib/Elements/Three-Phase Parallel RLC Branch  LConnTagsString=A|B|C  RConnTagsString=A|B|C  BranchType=RL  Resistance=0.0493  Inductance=0.0251  Capacitance=1e-6  Measurements=None
      settings: SourceProductName=Simscape Power Systems  SourceProductBaseCode=PS
  Line 9-10 : powerlib/Elements/Three-Phase Parallel RLC Branch  LConnTagsString=A|B|C  RConnTagsString=A|B|C  BranchType=RL  Resistance=0.819  Inductance=0.2707  Capacitance=1e-6  Measurements=None
      settings: SourceProductName=Simscape Power Systems  SourceProductBaseCode=PS
  Line 9-53 : powerlib/Elements/Three-Phase Parallel RLC Branch  LConnTagsString=A|B|C  RConnTagsString=A|B|C  BranchType=RL  Resistance=0.174  Inductance=0.0886  Capacitance=1e-6  Measurements=None
      settings: SourceProductName=Simscape Power Systems  SourceProductBaseCode=PS
  Load Flow Bus : powerlib/Measurements/Load Flow Bus  LConnTagsString=a  Phases=single  Connectors=on one side  ID=BUS_1  Vbase=13.8e3  Vref=1  Vangle=0  VLF=1  VLFb=1  VLFc=1  angleLF=0  angleLFb=0  angleLFc=0
      settings: SourceProductName=Simscape Power Systems
  Load Flow Bus1 : powerlib/Measurements/Load Flow Bus  LConnTagsString=a  Phases=single  Connectors=on one side  ID=BUS_2  Vbase=13.8e3  Vref=1  Vangle=0  VLF=1  VLFb=1  VLFc=1  angleLF=0  angleLFb=0  angleLFc=0
      settings: SourceProductName=Simscape Power Systems
  Load Flow Bus10 : powerlib/Measurements/Load Flow Bus  LConnTagsString=a  Phases=single  Connectors=on one side  ID=BUS_11  Vbase=13.8e3  Vref=1  Vangle=0  VLF=1  VLFb=1  VLFc=1  angleLF=0  angleLFb=0  angleLFc=0
      settings: SourceProductName=Simscape Power Systems
  Load Flow Bus11 : powerlib/Measurements/Load Flow Bus  LConnTagsString=a  Phases=single  Connectors=on one side  ID=BUS_12  Vbase=13.8e3  Vref=1  Vangle=0  VLF=1  VLFb=1  VLFc=1  angleLF=0  angleLFb=0  angleLFc=0
      settings: SourceProductName=Simscape Power Systems
  Load Flow Bus12 : powerlib/Measurements/Load Flow Bus  LConnTagsString=a  Phases=single  Connectors=on one side  ID=BUS_13  Vbase=13.8e3  Vref=1  Vangle=0  VLF=1  VLFb=1  VLFc=1  angleLF=0  angleLFb=0  angleLFc=0
      settings: SourceProductName=Simscape Power Systems
  Load Flow Bus13 : powerlib/Measurements/Load Flow Bus  LConnTagsString=a  Phases=single  Connectors=on one side  ID=BUS_14  Vbase=13.8e3  Vref=1  Vangle=0  VLF=1  VLFb=1  VLFc=1  angleLF=0  angleLFb=0  angleLFc=0
      settings: SourceProductName=Simscape Power Systems
  Load Flow Bus14 : powerlib/Measurements/Load Flow Bus  LConnTagsString=a  Phases=single  Connectors=on one side  ID=BUS_15  Vbase=13.8e3  Vref=1  Vangle=0  VLF=1  VLFb=1  VLFc=1  angleLF=0  angleLFb=0  angleLFc=0
      settings: SourceProductName=Simscape Power Systems
  Load Flow Bus15 : powerlib/Measurements/Load Flow Bus  LConnTagsString=a  Phases=single  Connectors=on one side  ID=BUS_16  Vbase=13.8e3  Vref=1  Vangle=0  VLF=1  VLFb=1  VLFc=1  angleLF=0  angleLFb=0  angleLFc=0
      settings: SourceProductName=Simscape Power Systems
  Load Flow Bus16 : powerlib/Measurements/Load Flow Bus  LConnTagsString=a  Phases=single  Connectors=on one side  ID=BUS_17  Vbase=13.8e3  Vref=1  Vangle=0  VLF=1  VLFb=1  VLFc=1  angleLF=0  angleLFb=0  angleLFc=0
      settings: SourceProductName=Simscape Power Systems
  Load Flow Bus17 : powerlib/Measurements/Load Flow Bus  LConnTagsString=a  Phases=single  Connectors=on one side  ID=BUS_18  Vbase=13.8e3  Vref=1  Vangle=0  VLF=1  VLFb=1  VLFc=1  angleLF=0  angleLFb=0  angleLFc=0
      settings: SourceProductName=Simscape Power Systems
  Load Flow Bus18 : powerlib/Measurements/Load Flow Bus  LConnTagsString=a  Phases=single  Connectors=on one side  ID=BUS_19  Vbase=13.8e3  Vref=1  Vangle=0  VLF=1  VLFb=1  VLFc=1  angleLF=0  angleLFb=0  angleLFc=0
      settings: SourceProductName=Simscape Power Systems
  Load Flow Bus19 : powerlib/Measurements/Load Flow Bus  LConnTagsString=a  Phases=single  Connectors=on one side  ID=BUS_20  Vbase=13.8e3  Vref=1  Vangle=0  VLF=1  VLFb=1  VLFc=1  angleLF=0  angleLFb=0  angleLFc=0
      settings: SourceProductName=Simscape Power Systems
  Load Flow Bus2 : powerlib/Measurements/Load Flow Bus  LConnTagsString=a  Phases=single  Connectors=on one side  ID=BUS_3  Vbase=13.8e3  Vref=1  Vangle=0  VLF=1  VLFb=1  VLFc=1  angleLF=0  angleLFb=0  angleLFc=0
      settings: SourceProductName=Simscape Power Systems
  Load Flow Bus20 : powerlib/Measurements/Load Flow Bus  LConnTagsString=a  Phases=single  Connectors=on one side  ID=BUS_21  Vbase=13.8e3  Vref=1  Vangle=0  VLF=1  VLFb=1  VLFc=1  angleLF=0  angleLFb=0  angleLFc=0
      settings: SourceProductName=Simscape Power Systems
  Load Flow Bus21 : powerlib/Measurements/Load Flow Bus  LConnTagsString=a  Phases=single  Connectors=on one side  ID=BUS_22  Vbase=13.8e3  Vref=1  Vangle=0  VLF=1  VLFb=1  VLFc=1  angleLF=0  angleLFb=0  angleLFc=0
      settings: SourceProductName=Simscape Power Systems
  Load Flow Bus22 : powerlib/Measurements/Load Flow Bus  LConnTagsString=a  Phases=single  Connectors=on one side  ID=BUS_23  Vbase=13.8e3  Vref=1  Vangle=0  VLF=1  VLFb=1  VLFc=1  angleLF=0  angleLFb=0  angleLFc=0
      settings: SourceProductName=Simscape Power Systems
  Load Flow Bus23 : powerlib/Measurements/Load Flow Bus  LConnTagsString=a  Phases=single  Connectors=on one side  ID=BUS_24  Vbase=13.8e3  Vref=1  Vangle=0  VLF=1  VLFb=1  VLFc=1  angleLF=0  angleLFb=0  angleLFc=0
      settings: SourceProductName=Simscape Power Systems
  Load Flow Bus24 : powerlib/Measurements/Load Flow Bus  LConnTagsString=a  Phases=single  Connectors=on one side  ID=BUS_25  Vbase=13.8e3  Vref=1  Vangle=0  VLF=1  VLFb=1  VLFc=1  angleLF=0  angleLFb=0  angleLFc=0
      settings: SourceProductName=Simscape Power Systems
  Load Flow Bus25 : powerlib/Measurements/Load Flow Bus  LConnTagsString=a  Phases=single  Connectors=on one side  ID=BUS_26  Vbase=13.8e3  Vref=1  Vangle=0  VLF=1  VLFb=1  VLFc=1  angleLF=0  angleLFb=0  angleLFc=0
      settings: SourceProductName=Simscape Power Systems
  Load Flow Bus26 : powerlib/Measurements/Load Flow Bus  LConnTagsString=a  Phases=single  Connectors=on one side  ID=BUS_27  Vbase=13.8e3  Vref=1  Vangle=0  VLF=1  VLFb=1  VLFc=1  angleLF=0  angleLFb=0  angleLFc=0
      settings: SourceProductName=Simscape Power Systems
  Load Flow Bus27 : powerlib/Measurements/Load Flow Bus  LConnTagsString=a  Phases=single  Connectors=on one side  ID=BUS_28  Vbase=13.8e3  Vref=1  Vangle=0  VLF=1  VLFb=1  VLFc=1  angleLF=0  angleLFb=0  angleLFc=0
      settings: SourceProductName=Simscape Power Systems
  Load Flow Bus28 : powerlib/Measurements/Load Flow Bus  LConnTagsString=a  Phases=single  Connectors=on one side  ID=BUS_29  Vbase=13.8e3  Vref=1  Vangle=0  VLF=1  VLFb=1  VLFc=1  angleLF=0  angleLFb=0  angleLFc=0
      settings: SourceProductName=Simscape Power Systems
  Load Flow Bus29 : powerlib/Measurements/Load Flow Bus  LConnTagsString=a  Phases=single  Connectors=on one side  ID=BUS_30  Vbase=13.8e3  Vref=1  Vangle=0  VLF=1  VLFb=1  VLFc=1  angleLF=0  angleLFb=0  angleLFc=0
      settings: SourceProductName=Simscape Power Systems
  Load Flow Bus3 : powerlib/Measurements/Load Flow Bus  LConnTagsString=a  Phases=single  Connectors=on one side  ID=BUS_4  Vbase=13.8e3  Vref=1  Vangle=0  VLF=1  VLFb=1  VLFc=1  angleLF=0  angleLFb=0  angleLFc=0
      settings: SourceProductName=Simscape Power Systems
  Load Flow Bus30 : powerlib/Measurements/Load Flow Bus  LConnTagsString=a  Phases=single  Connectors=on one side  ID=BUS_31  Vbase=13.8e3  Vref=1  Vangle=0  VLF=1  VLFb=1  VLFc=1  angleLF=0  angleLFb=0  angleLFc=0
      settings: SourceProductName=Simscape Power Systems
  Load Flow Bus31 : powerlib/Measurements/Load Flow Bus  LConnTagsString=a  Phases=single  Connectors=on one side  ID=BUS_32  Vbase=13.8e3  Vref=1  Vangle=0  VLF=1  VLFb=1  VLFc=1  angleLF=0  angleLFb=0  angleLFc=0
      settings: SourceProductName=Simscape Power Systems
  Load Flow Bus32 : powerlib/Measurements/Load Flow Bus  LConnTagsString=a  Phases=single  Connectors=on one side  ID=BUS_33  Vbase=13.8e3  Vref=1  Vangle=0  VLF=1  VLFb=1  VLFc=1  angleLF=0  angleLFb=0  angleLFc=0
      settings: SourceProductName=Simscape Power Systems
  Load Flow Bus33 : powerlib/Measurements/Load Flow Bus  LConnTagsString=a  Phases=single  Connectors=on one side  ID=BUS_34  Vbase=13.8e3  Vref=1  Vangle=0  VLF=1  VLFb=1  VLFc=1  angleLF=0  angleLFb=0  angleLFc=0
      settings: SourceProductName=Simscape Power Systems
  Load Flow Bus34 : powerlib/Measurements/Load Flow Bus  LConnTagsString=a  Phases=single  Connectors=on one side  ID=BUS_35  Vbase=13.8e3  Vref=1  Vangle=0  VLF=1  VLFb=1  VLFc=1  angleLF=0  angleLFb=0  angleLFc=0
      settings: SourceProductName=Simscape Power Systems
  Load Flow Bus35 : powerlib/Measurements/Load Flow Bus  LConnTagsString=a  Phases=single  Connectors=on one side  ID=BUS_36  Vbase=13.8e3  Vref=1  Vangle=0  VLF=1  VLFb=1  VLFc=1  angleLF=0  angleLFb=0  angleLFc=0
      settings: SourceProductName=Simscape Power Systems
  Load Flow Bus36 : powerlib/Measurements/Load Flow Bus  LConnTagsString=a  Phases=single  Connectors=on one side  ID=BUS_37  Vbase=13.8e3  Vref=1  Vangle=0  VLF=1  VLFb=1  VLFc=1  angleLF=0  angleLFb=0  angleLFc=0
      settings: SourceProductName=Simscape Power Systems
  Load Flow Bus37 : powerlib/Measurements/Load Flow Bus  LConnTagsString=a  Phases=single  Connectors=on one side  ID=BUS_38  Vbase=13.8e3  Vref=1  Vangle=0  VLF=1  VLFb=1  VLFc=1  angleLF=0  angleLFb=0  angleLFc=0
      settings: SourceProductName=Simscape Power Systems
  Load Flow Bus38 : powerlib/Measurements/Load Flow Bus  LConnTagsString=a  Phases=single  Connectors=on one side  ID=BUS_39  Vbase=13.8e3  Vref=1  Vangle=0  VLF=1  VLFb=1  VLFc=1  angleLF=0  angleLFb=0  angleLFc=0
      settings: SourceProductName=Simscape Power Systems
  Load Flow Bus39 : powerlib/Measurements/Load Flow Bus  LConnTagsString=a  Phases=single  Connectors=on one side  ID=BUS_40  Vbase=13.8e3  Vref=1  Vangle=0  VLF=1  VLFb=1  VLFc=1  angleLF=0  angleLFb=0  angleLFc=0
      settings: SourceProductName=Simscape Power Systems
  Load Flow Bus4 : powerlib/Measurements/Load Flow Bus  LConnTagsString=a  Phases=single  Connectors=on one side  ID=BUS_5  Vbase=13.8e3  Vref=1  Vangle=0  VLF=1  VLFb=1  VLFc=1  angleLF=0  angleLFb=0  angleLFc=0
      settings: SourceProductName=Simscape Power Systems
  Load Flow Bus40 : powerlib/Measurements/Load Flow Bus  LConnTagsString=a  Phases=single  Connectors=on one side  ID=BUS_41  Vbase=13.8e3  Vref=1  Vangle=0  VLF=1  VLFb=1  VLFc=1  angleLF=0  angleLFb=0  angleLFc=0
      settings: SourceProductName=Simscape Power Systems
  Load Flow Bus41 : powerlib/Measurements/Load Flow Bus  LConnTagsString=a  Phases=single  Connectors=on one side  ID=BUS_42  Vbase=13.8e3  Vref=1  Vangle=0  VLF=1  VLFb=1  VLFc=1  angleLF=0  angleLFb=0  angleLFc=0
      settings: SourceProductName=Simscape Power Systems
  Load Flow Bus42 : powerlib/Measurements/Load Flow Bus  LConnTagsString=a  Phases=single  Connectors=on one side  ID=BUS_43  Vbase=13.8e3  Vref=1  Vangle=0  VLF=1  VLFb=1  VLFc=1  angleLF=0  angleLFb=0  angleLFc=0
      settings: SourceProductName=Simscape Power Systems
  Load Flow Bus43 : powerlib/Measurements/Load Flow Bus  LConnTagsString=a  Phases=single  Connectors=on one side  ID=BUS_44  Vbase=13.8e3  Vref=1  Vangle=0  VLF=1  VLFb=1  VLFc=1  angleLF=0  angleLFb=0  angleLFc=0
      settings: SourceProductName=Simscape Power Systems
  Load Flow Bus44 : powerlib/Measurements/Load Flow Bus  LConnTagsString=a  Phases=single  Connectors=on one side  ID=BUS_45  Vbase=13.8e3  Vref=1  Vangle=0  VLF=1  VLFb=1  VLFc=1  angleLF=0  angleLFb=0  angleLFc=0
      settings: SourceProductName=Simscape Power Systems
  Load Flow Bus45 : powerlib/Measurements/Load Flow Bus  LConnTagsString=a  Phases=single  Connectors=on one side  ID=BUS_46  Vbase=13.8e3  Vref=1  Vangle=0  VLF=1  VLFb=1  VLFc=1  angleLF=0  angleLFb=0  angleLFc=0
      settings: SourceProductName=Simscape Power Systems
  Load Flow Bus46 : powerlib/Measurements/Load Flow Bus  LConnTagsString=a  Phases=single  Connectors=on one side  ID=BUS_47  Vbase=13.8e3  Vref=1  Vangle=0  VLF=1  VLFb=1  VLFc=1  angleLF=0  angleLFb=0  angleLFc=0
      settings: SourceProductName=Simscape Power Systems
  Load Flow Bus47 : powerlib/Measurements/Load Flow Bus  LConnTagsString=a  Phases=single  Connectors=on one side  ID=BUS_48  Vbase=13.8e3  Vref=1  Vangle=0  VLF=1  VLFb=1  VLFc=1  angleLF=0  angleLFb=0  angleLFc=0
      settings: SourceProductName=Simscape Power Systems
  Load Flow Bus48 : powerlib/Measurements/Load Flow Bus  LConnTagsString=a  Phases=single  Connectors=on one side  ID=BUS_49  Vbase=13.8e3  Vref=1  Vangle=0  VLF=1  VLFb=1  VLFc=1  angleLF=0  angleLFb=0  angleLFc=0
      settings: SourceProductName=Simscape Power Systems
  Load Flow Bus49 : powerlib/Measurements/Load Flow Bus  LConnTagsString=a  Phases=single  Connectors=on one side  ID=BUS_50  Vbase=13.8e3  Vref=1  Vangle=0  VLF=1  VLFb=1  VLFc=1  angleLF=0  angleLFb=0  angleLFc=0
      settings: SourceProductName=Simscape Power Systems
  Load Flow Bus5 : powerlib/Measurements/Load Flow Bus  LConnTagsString=a  Phases=single  Connectors=on one side  ID=BUS_6  Vbase=13.8e3  Vref=1  Vangle=0  VLF=1  VLFb=1  VLFc=1  angleLF=0  angleLFb=0  angleLFc=0
      settings: SourceProductName=Simscape Power Systems
  Load Flow Bus50 : powerlib/Measurements/Load Flow Bus  LConnTagsString=a  Phases=single  Connectors=on one side  ID=BUS_51  Vbase=13.8e3  Vref=1  Vangle=0  VLF=1  VLFb=1  VLFc=1  angleLF=0  angleLFb=0  angleLFc=0
      settings: SourceProductName=Simscape Power Systems
  Load Flow Bus51 : powerlib/Measurements/Load Flow Bus  LConnTagsString=a  Phases=single  Connectors=on one side  ID=BUS_52  Vbase=13.8e3  Vref=1  Vangle=0  VLF=1  VLFb=1  VLFc=1  angleLF=0  angleLFb=0  angleLFc=0
      settings: SourceProductName=Simscape Power Systems
  Load Flow Bus52 : powerlib/Measurements/Load Flow Bus  LConnTagsString=a  Phases=single  Connectors=on one side  ID=BUS_53  Vbase=13.8e3  Vref=1  Vangle=0  VLF=1  VLFb=1  VLFc=1  angleLF=0  angleLFb=0  angleLFc=0
      settings: SourceProductName=Simscape Power Systems
  Load Flow Bus53 : powerlib/Measurements/Load Flow Bus  LConnTagsString=a  Phases=single  Connectors=on one side  ID=BUS_54  Vbase=13.8e3  Vref=1  Vangle=0  VLF=1  VLFb=1  VLFc=1  angleLF=0  angleLFb=0  angleLFc=0
      settings: SourceProductName=Simscape Power Systems
  Load Flow Bus54 : powerlib/Measurements/Load Flow Bus  LConnTagsString=a  Phases=single  Connectors=on one side  ID=BUS_55  Vbase=13.8e3  Vref=1  Vangle=0  VLF=1  VLFb=1  VLFc=1  angleLF=0  angleLFb=0  angleLFc=0
      settings: SourceProductName=Simscape Power Systems
  Load Flow Bus55 : powerlib/Measurements/Load Flow Bus  LConnTagsString=a  Phases=single  Connectors=on one side  ID=BUS_56  Vbase=13.8e3  Vref=1  Vangle=0  VLF=1  VLFb=1  VLFc=1  angleLF=0  angleLFb=0  angleLFc=0
      settings: SourceProductName=Simscape Power Systems
  Load Flow Bus56 : powerlib/Measurements/Load Flow Bus  LConnTagsString=a  Phases=single  Connectors=on one side  ID=BUS_57  Vbase=13.8e3  Vref=1  Vangle=0  VLF=1  VLFb=1  VLFc=1  angleLF=0  angleLFb=0  angleLFc=0
      settings: SourceProductName=Simscape Power Systems
  Load Flow Bus57 : powerlib/Measurements/Load Flow Bus  LConnTagsString=a  Phases=single  Connectors=on one side  ID=BUS_58  Vbase=13.8e3  Vref=1  Vangle=0  VLF=1  VLFb=1  VLFc=1  angleLF=0  angleLFb=0  angleLFc=0
      settings: SourceProductName=Simscape Power Systems
  Load Flow Bus58 : powerlib/Measurements/Load Flow Bus  LConnTagsString=a  Phases=single  Connectors=on one side  ID=BUS_59  Vbase=13.8e3  Vref=1  Vangle=0  VLF=1  VLFb=1  VLFc=1  angleLF=0  angleLFb=0  angleLFc=0
      settings: SourceProductName=Simscape Power Systems
  Load Flow Bus59 : powerlib/Measurements/Load Flow Bus  LConnTagsString=a  Phases=single  Connectors=on one side  ID=BUS_60  Vbase=13.8e3  Vref=1  Vangle=0  VLF=1  VLFb=1  VLFc=1  angleLF=0  angleLFb=0  angleLFc=0
      settings: SourceProductName=Simscape Power Systems
  Load Flow Bus6 : powerlib/Measurements/Load Flow Bus  LConnTagsString=a  Phases=single  Connectors=on one side  ID=BUS_7  Vbase=13.8e3  Vref=1  Vangle=0  VLF=1  VLFb=1  VLFc=1  angleLF=0  angleLFb=0  angleLFc=0
      settings: SourceProductName=Simscape Power Systems
  Load Flow Bus60 : powerlib/Measurements/Load Flow Bus  LConnTagsString=a  Phases=single  Connectors=on one side  ID=BUS_61  Vbase=13.8e3  Vref=1  Vangle=0  VLF=1  VLFb=1  VLFc=1  angleLF=0  angleLFb=0  angleLFc=0
      settings: SourceProductName=Simscape Power Systems
  Load Flow Bus61 : powerlib/Measurements/Load Flow Bus  LConnTagsString=a  Phases=single  Connectors=on one side  ID=BUS_62  Vbase=13.8e3  Vref=1  Vangle=0  VLF=1  VLFb=1  VLFc=1  angleLF=0  angleLFb=0  angleLFc=0
      settings: SourceProductName=Simscape Power Systems
  Load Flow Bus62 : powerlib/Measurements/Load Flow Bus  LConnTagsString=a  Phases=single  Connectors=on one side  ID=BUS_63  Vbase=13.8e3  Vref=1  Vangle=0  VLF=1  VLFb=1  VLFc=1  angleLF=0  angleLFb=0  angleLFc=0
      settings: SourceProductName=Simscape Power Systems
  Load Flow Bus63 : powerlib/Measurements/Load Flow Bus  LConnTagsString=a  Phases=single  Connectors=on one side  ID=BUS_64  Vbase=13.8e3  Vref=1  Vangle=0  VLF=1  VLFb=1  VLFc=1  angleLF=0  angleLFb=0  angleLFc=0
      settings: SourceProductName=Simscape Power Systems
  Load Flow Bus64 : powerlib/Measurements/Load Flow Bus  LConnTagsString=a  Phases=single  Connectors=on one side  ID=BUS_65  Vbase=13.8e3  Vref=1  Vangle=0  VLF=1  VLFb=1  VLFc=1  angleLF=0  angleLFb=0  angleLFc=0
      settings: SourceProductName=Simscape Power Systems
  Load Flow Bus65 : powerlib/Measurements/Load Flow Bus  LConnTagsString=a  Phases=single  Connectors=on one side  ID=BUS_66  Vbase=13.8e3  Vref=1  Vangle=0  VLF=1  VLFb=1  VLFc=1  angleLF=0  angleLFb=0  angleLFc=0
      settings: SourceProductName=Simscape Power Systems
  Load Flow Bus66 : powerlib/Measurements/Load Flow Bus  LConnTagsString=a  Phases=single  Connectors=on one side  ID=BUS_67  Vbase=13.8e3  Vref=1  Vangle=0  VLF=1  VLFb=1  VLFc=1  angleLF=0  angleLFb=0  angleLFc=0
      settings: SourceProductName=Simscape Power Systems
  Load Flow Bus67 : powerlib/Measurements/Load Flow Bus  LConnTagsString=a  Phases=single  Connectors=on one side  ID=BUS_68  Vbase=13.8e3  Vref=1  Vangle=0  VLF=1  VLFb=1  VLFc=1  angleLF=0  angleLFb=0  angleLFc=0
      settings: SourceProductName=Simscape Power Systems
  Load Flow Bus68 : powerlib/Measurements/Load Flow Bus  LConnTagsString=a  Phases=single  Connectors=on one side  ID=BUS_69  Vbase=13.8e3  Vref=1  Vangle=0  VLF=1  VLFb=1  VLFc=1  angleLF=0  angleLFb=0  angleLFc=0
      settings: SourceProductName=Simscape Power Systems
  Load Flow Bus7 : powerlib/Measurements/Load Flow Bus  LConnTagsString=a  Phases=single  Connectors=on one side  ID=BUS_8  Vbase=13.8e3  Vref=1  Vangle=0  VLF=1  VLFb=1  VLFc=1  angleLF=0  angleLFb=0  angleLFc=0
      settings: SourceProductName=Simscape Power Systems
  Load Flow Bus8 : powerlib/Measurements/Load Flow Bus  LConnTagsString=a  Phases=single  Connectors=on one side  ID=BUS_9  Vbase=13.8e3  Vref=1  Vangle=0  VLF=1  VLFb=1  VLFc=1  angleLF=0  angleLFb=0  angleLFc=0
      settings: SourceProductName=Simscape Power Systems
  Load Flow Bus9 : powerlib/Measurements/Load Flow Bus  LConnTagsString=a  Phases=single  Connectors=on one side  ID=BUS_10  Vbase=13.8e3  Vref=1  Vangle=0  VLF=1  VLFb=1  VLFc=1  angleLF=0  angleLFb=0  angleLFc=0
      settings: SourceProductName=Simscape Power Systems
  Multimeter : powerlib/Measurements/Multimeter  PhasorSimulation=off  OutputType=Complex  sel=[1 2 3 4 5 6]  L=6  Gain=[1 1 1 1 1 1]  yselected="{'Uag: 2 MW  11 kV','Ubg: 2 MW  11 kV','Ucg: 2 MW  11 kV','Iag: 2 MW  11 kV','Ibg: 2 MW  11 kV','Icg: 2 MW  11 kV'};"  PSBOutputType=1  PSBequivalent=0  AxesSetting=[0,0.1,-100,100]  Display=0  SavedBlockNames=-11
  Scope : Scope  NumInputPorts=2
  Three-Phase Parallel RLC Load23 : powerlib/Elements/Three-Phase Parallel RLC Load  LConnTagsString=A|B|C  Configuration=Y (grounded)  NominalVoltage=11e3  Vabc=[1e3 1e3 1e3]  Vabcp=[1e3 1e3 1e3]  NominalFrequency=50  UnbalancedPower=off  ActivePower=14e3  InductivePower=100  CapacitivePower=0  Pabc=[10e3 9e3 11e3]  QLabc=[100 90 110]  QCabc=[100 90 110]  Pabcp=[10e3 9e3 11e3]  QLabcp=[100 90 110]  QCabcp=[100 90 110]  Measurements=None  LoadType=constant Z
  Three-Phase Parallel RLC Load42 : powerlib/Elements/Three-Phase Parallel RLC Load  LConnTagsString=A|B|C  Configuration=Y (grounded)  NominalVoltage=11e3  Vabc=[1e3 1e3 1e3]  Vabcp=[1e3 1e3 1e3]  NominalFrequency=50  UnbalancedPower=off  ActivePower=6e3  InductivePower=100  CapacitivePower=100  Pabc=[10e3 9e3 11e3]  QLabc=[100 90 110]  QCabc=[100 90 110]  Pabcp=[10e3 9e3 11e3]  QLabcp=[100 90 110]  QCabcp=[100 90 110]  Measurements=None  LoadType=constant Z
  powergui : powerlib/powergui  Priority=1  SimulationMode=Discrete  SampleTime=50e-6  frequency=60  Iterations=50  frequencyindice=50  Pbase=100e6  ErrMax=1e-4  UnitsV=kV  UnitsW=MW  buscounter=0  FunctionMessages=off  echomessages=off  EnableUseOfTLC=off  CurrentSourceSwitches=off  DisableSnubberDevices=off  DisableRonSwitches=off  DisableVfSwitches=off  DisplayEquations=off  SolverType=Tustin  Interpol=off  ExternalGateDelay=off  methode=off  Ts=100  x0status=zero  SPID=on  SwTol=0  HookPort=off  RestoreLinks=warning  ResistiveCurrentMeasurement=off  Frange=[0:2:500]  Ylog=off  Xlog=on  ShowGrid=off  save=off  variable=ZData  structure=logsout  ZoomFFT=off  StartTime=0.0  cycles=1  DisplayStyle=1  fundamental=60  FreqAxis=off  MaxFrequency=1000  frequencyindicesteady=1  RmsSteady=1  display=off
  wires:
  Multimeter/1 -> Demux/1
  Demux/1 -> Scope/1
  Demux/2 -> Scope/2
  connections:
  2 6 kW 11 kV/LConn2 -- BUS 44/RConn2 -- Line 44-45/LConn2
  Load Flow Bus59/LConn1 -- BUS 60/RConn3 -- Line 60-61/LConn3
  Line 11-66/LConn2 -- 145 kW 11 kV/LConn2 -- Line 11-12/LConn2 -- BUS 11/RConn2
  BUS 35/RConn3 -- Load Flow Bus34/LConn1 -- Three-Phase Parallel RLC Load42/LConn3
  Line 64-65/LConn1 -- 227 kW 11 kV/LConn1 -- BUS 64/RConn1
  Line 45-46/LConn2 -- 39.2 kW 11 kV/LConn2 -- BUS 45/RConn2
  5 kW 11 kV/LConn2 -- BUS 22/RConn2 -- Line 22-23/LConn2
  26.4 kW 11 kV/LConn3 -- BUS 54/RConn3 -- Line 54-55/LConn3 -- Load Flow Bus53/LConn1
  BUS 12/RConn2 -- Line 12-68/LConn2 -- Line 12-13/LConn2
  Line 8-51/LConn3 -- Load Flow Bus7/LConn1 -- BUS 8/RConn3 -- Line 8-9/LConn3
  60 kW 11 kV/LConn2 -- BUS 17/RConn2 -- Line 17-18/LConn2
  60 kW 11 kV/LConn1 -- BUS 17/RConn1 -- Line 17-18/LConn1
  39.2 kW 11 kV/LConn3 -- Line 45-46/LConn3 -- BUS 45/RConn3 -- Load Flow Bus44/LConn1
  BUS 12/RConn1 -- Line 12-68/LConn1 -- Line 12-13/LConn1
  Line 12-68/LConn3 -- Load Flow Bus11/LConn1 -- BUS 12/RConn3 -- Line 12-13/LConn3
  18 kW 11 kV/LConn1 -- BUS 66/RConn1 -- Line 66-67/LConn1
  BUS 69/RConn3 -- Load Flow Bus68/LConn1 -- 3 28 kW 11 kV/LConn3
  Load Flow Bus/LConn1 -- Line 1-2/LConn3 -- BUS 1/RConn3
  5 kW 11 kV/LConn1 -- BUS 22/RConn1 -- Line 22-23/LConn1
  3 30 kW 11 kV/LConn1 -- BUS 37/RConn1 -- Line 37-38/LConn1
  5 kW 11 kV/LConn3 -- BUS 22/RConn3 -- Line 22-23/LConn3 -- Load Flow Bus21/LConn1
  Load Flow Bus41/LConn1 -- Line 42-43/LConn3 -- BUS 42/RConn3
  4 MW 11 kV/LConn1 -- BUS 26/RConn1 -- 14 kW 11 kV/LConn1 -- Line 26-27/LConn1
  30 kW 11 kV/LConn2 -- Line 9-53/LConn2 -- BUS 9/RConn2 -- Line 9-10/LConn2
  100 kW 11 kV/LConn3 -- BUS 59/RConn3 -- Line 59-60/LConn3 -- Load Flow Bus58/LConn1
  30 kW 11 kV/LConn3 -- Line 10-11/LConn3 -- BUS 10/RConn3 -- Load Flow Bus9/LConn1
  75 kW 11 kV/LConn2 -- Line 8-9/RConn2 -- BUS 9/LConn2
  BUS 33/RConn1 -- 2 14 kW 11 kV/LConn1 -- Line 33-34/LConn1
  Load Flow Bus26/LConn1 -- BUS 27/RConn3 -- Three-Phase Parallel RLC Load23/LConn3
  Load Flow Bus4/LConn1 -- BUS 5/RConn3 -- Line 5-6/LConn3
  BUS 48/RConn2 -- 79 kW 11 kV/LConn2 -- Line 48-49/LConn2
  Load Flow Bus61/LConn1 -- 32 kW 11 kV/LConn3 -- BUS 62/RConn3 -- Line 62-63/LConn3
  BUS 7/RConn2 -- 40 kW 11 kV/LConn2 -- Line 7-8/LConn2
  BUS 53/RConn1 -- 43.5 kW 11 kV/LConn1 -- Line 53-54/LConn1
  BUS 26/RConn3 -- 4 MW 11 kV/LConn3 -- Load Flow Bus25/LConn1 -- Line 26-27/LConn3 -- 14 kW 11 kV/LConn3
  Line 40-41/LConn2 -- 2 24 kW 11 kV/LConn2 -- BUS 40/RConn2
  BUS 37/RConn3 -- 3 30 kW 11 kV/LConn3 -- Line 37-38/LConn3 -- Load Flow Bus36/LConn1
  Load Flow Bus60/LConn1 -- 1244 kW 11 kV/LConn3 -- Line 61-62/LConn3 -- BUS 61/RConn3
  2 28 kW 11 kV/LConn1 -- BUS 68/RConn1 -- Line 68-69/LConn1
  Load Flow Bus37/LConn1 -- BUS 38/RConn3 -- Line 38-39/LConn3
  Line 31-32/LConn3 -- Load Flow Bus30/LConn1 -- BUS 31/RConn3
  Line 40-41/LConn1 -- 2 24 kW 11 kV/LConn1 -- BUS 40/RConn1
  BUS 47/RConn3 -- Load Flow Bus46/LConn1 -- Line 47-48/LConn3
  3 30 kW 11 kV/LConn2 -- BUS 37/RConn2 -- Line 37-38/LConn2
  Load Flow Bus39/LConn1 -- 2 24 kW 11 kV/LConn3 -- BUS 40/RConn3 -- Line 40-41/LConn3
  1.2 kW 11 kV/LConn1 -- BUS 41/RConn1 -- Line 41-42/LConn1
  1244 kW 11 kV/LConn1 -- BUS 61/RConn1 -- Line 61-62/LConn1
  Load Flow Bus64/LConn1 -- BUS 65/RConn3 -- 59 kW 11 kV/LConn3
  2 14 kW 11 kV/LConn2 -- BUS 33/RConn2 -- Line 33-34/LConn2
  384.7 kW 11 kV/LConn1 -- BUS 49/RConn1 -- Line 49-50/LConn1
  28 kW 11 kV/LConn1 -- BUS 23/RConn1 -- Line 23-24/LConn1
  Line 8-51/LConn1 -- BUS 8/RConn1 -- Line 8-9/LConn1
  BUS 21/RConn2 -- 114 kW 11 kV/LConn2 -- Line 21-22/LConn2
  Line 11-66/LConn1 -- 145 kW 11 kV/LConn1 -- Line 11-12/LConn1 -- BUS 11/RConn1
  1 kW 11 kV/LConn2 -- BUS 20/RConn2 -- Line 20-21/LConn2
  8 kW 11 kV/LConn2 -- BUS 13/RConn2 -- Line 13-14/LConn2
  Load Flow Bus32/LConn1 -- 2 14 kW 11 kV/LConn3 -- Line 33-34/LConn3 -- BUS 33/RConn3
  24 kW 11 kV/LConn3 -- BUS 39/RConn3 -- Line 39-40/LConn3 -- Load Flow Bus38/LConn1
  384.7 kW 11 kV/LConn2 -- BUS 49/RConn2 -- Line 49-50/LConn2
  40 kW 11 kV/LConn1 -- BUS 7/RConn1 -- Line 7-8/LConn1
  Load Flow Bus57/LConn1 -- BUS 58/RConn3 -- Line 58-59/LConn3
  Load Flow Bus13/LConn1 -- 2 8 kW 11 kV/LConn3 -- Line 14-15/LConn3 -- BUS 14/RConn3
  2 26 kW 11 kV/LConn1 -- BUS 29/RConn1 -- Line 29-30/LConn1
  6 kW 11 kV/LConn2 -- BUS 43/RConn2 -- Line 43-44/LConn2
  Load Flow Bus62/LConn1 -- BUS 63/RConn3 -- Line 63-64/LConn3
  BUS 32/RConn3 -- Load Flow Bus31/LConn1 -- Line 32-33/LConn3
  BUS 19/RConn3 -- Load Flow Bus18/LConn1 -- Line 19-20/LConn3
  BUS 23/RConn3 -- 28 kW 11 kV/LConn3 -- Line 23-24/LConn3 -- Load Flow Bus22/LConn1
  Load Flow Bus54/LConn1 -- BUS 55/RConn3 -- Line 55-56/LConn3
  Load Flow Bus5/LConn1 -- BUS 6/RConn3 -- Line 6-7/LConn3
  Load Flow Bus12/LConn1 -- 8 kW 11 kV/LConn3 -- Line 13-14/LConn3 -- BUS 13/RConn3
  Load Flow Bus10/LConn1 -- 145 kW 11 kV/LConn3 -- Line 11-12/LConn3 -- BUS 11/RConn3 -- Line 11-66/LConn3
  BUS 15/RConn3 -- Load Flow Bus14/LConn1 -- Line 15-16/LConn3
  BUS 61/RConn2 -- 1244 kW 11 kV/LConn2 -- Line 61-62/LConn2
  28 kW 11 kV/LConn2 -- BUS 23/RConn2 -- Line 23-24/LConn2
  Line 4-47/LConn1 -- Line 4-5/RConn1 -- BUS 5/LConn1
  2 MW 11 kV/LConn2 -- Line 3-4/RConn2 -- BUS 4/LConn2
  2 26 kW 11 kV/LConn3 -- BUS 29/RConn3 -- Line 29-30/LConn3 -- Load Flow Bus28/LConn1
  26.4 kW 11 kV/LConn1 -- BUS 54/RConn1 -- Line 54-55/LConn1
  BUS 18/RConn2 -- 2 60 kW 11 kV/LConn2 -- Line 18-19/LConn2
  Load Flow Bus27/LConn1 -- 26 kW 11 kV/LConn3 -- Line 28-29/LConn3 -- BUS 28/RConn3
  Line 4-47/LConn3 -- Line 4-5/RConn3 -- BUS 5/LConn3
  2 28 kW 11 kV/LConn2 -- BUS 68/RConn2 -- Line 68-69/LConn2
  Line 45-46/LConn1 -- 39.2 kW 11 kV/LConn1 -- BUS 45/RConn1
  Load Flow Bus49/LConn1 -- BUS 50/RConn3 -- 2 384.7 kW 11 kV/LConn3
  BUS 28/RConn2 -- 26 kW 11 kV/LConn2 -- Line 28-29/LConn2
  8 kW 11 kV/LConn1 -- BUS 13/RConn1 -- Line 13-14/LConn1
  2 30 kW 11 kV/LConn3 -- BUS 36/LConn3 -- Line 3-36/RConn3
  18 kW 11 kV/LConn3 -- BUS 66/RConn3 -- Line 66-67/LConn3 -- Load Flow Bus65/LConn1
  BUS 34/RConn1 -- 19.5 kW 11 kV/LConn1 -- Line 34-35/LConn1
  6 kW 11 kV/LConn1 -- BUS 43/RConn1 -- Line 43-44/LConn1
  24 kW 11 kV/LConn2 -- BUS 39/RConn2 -- Line 39-40/LConn2
  BUS 14/RConn2 -- 2 8 kW 11 kV/LConn2 -- Line 14-15/LConn2
  BUS 3/RConn1 -- Line 3-4/LConn1 -- Line 3-28/LConn1 -- Line 3-36/LConn1
  BUS 67/RConn3 -- Load Flow Bus66/LConn1 -- 2 18 kW 11 kV/LConn3
  Load Flow Bus51/LConn1 -- BUS 52/RConn3 -- 3.6 kW 11 kV/LConn3
  100 kW 11 kV/LConn1 -- BUS 59/RConn1 -- Line 59-60/LConn1
  Line 3-36/LConn2 -- Line 3-4/LConn2 -- Line 3-28/LConn2 -- BUS 3/RConn2
  19.5 kW 11 kV/LConn2 -- BUS 34/RConn2 -- Line 34-35/LConn2
  Line 3-36/RConn2 -- 2 30 kW 11 kV/LConn2 -- BUS 36/LConn2
  Line 3-28/LConn3 -- Load Flow Bus2/LConn1 -- Line 3-4/LConn3 -- Line 3-36/LConn3 -- BUS 3/RConn3
  Load Flow Bus50/LConn1 -- 40.5 kW 11 kV/LConn3 -- Line 51-52/LConn3 -- BUS 51/RConn3
  79 kW 11 kV/LConn1 -- BUS 48/RConn1 -- Line 48-49/LConn1
  Load Flow Bus48/LConn1 -- 384.7 kW 11 kV/LConn3 -- Line 49-50/LConn3 -- BUS 49/RConn3
  Load Flow Bus15/LConn1 -- BUS 16/RConn3 -- Line 16-17/LConn3
  Load Flow Bus63/LConn1 -- 227 kW 11 kV/LConn3 -- BUS 64/RConn3 -- Line 64-65/LConn3
  Load Flow Bus8/LConn1 -- Line 9-53/LConn3 -- BUS 9/RConn3 -- Line 9-10/LConn3 -- 30 kW 11 kV/LConn3
  Load Flow Bus33/LConn1 -- 19.5 kW 11 kV/LConn3 -- Line 34-35/LConn3 -- BUS 34/RConn3
  114 kW 11 kV/LConn1 -- BUS 21/RConn1 -- Line 21-22/LConn1
  Line 64-65/LConn2 -- 227 kW 11 kV/LConn2 -- BUS 64/RConn2
  BUS 28/RConn1 -- 26 kW 11 kV/LConn1 -- Line 28-29/LConn1
  Line 8-51/LConn2 -- BUS 8/RConn2 -- Line 8-9/LConn2
  BUS 9/LConn1 -- 75 kW 11 kV/LConn1 -- Line 8-9/RConn1
  Line 36-37/LConn3 -- Load Flow Bus35/LConn1 -- BUS 36/RConn3
  2 26 kW 11 kV/LConn2 -- BUS 29/RConn2 -- Line 29-30/LConn2
  Load Flow Bus23/LConn1 -- BUS 24/RConn3 -- Line 24-25/LConn3
  Line 62-63/LConn1 -- 32 kW 11 kV/LConn1 -- BUS 62/RConn1
  Line 4-47/LConn2 -- Line 4-5/RConn2 -- BUS 5/LConn2
  BUS 20/RConn3 -- 1 kW 11 kV/LConn3 -- Line 20-21/LConn3 -- Load Flow Bus19/LConn1
  26.4 kW 11 kV/LConn2 -- BUS 54/RConn2 -- Line 54-55/LConn2
  BUS 36/LConn1 -- 2 30 kW 11 kV/LConn1 -- Line 3-36/RConn1
  40.5 kW 11 kV/LConn2 -- Line 51-52/LConn2 -- BUS 51/RConn2
  1 kW 11 kV/LConn1 -- BUS 20/RConn1 -- Line 20-21/LConn1
  Load Flow Bus45/LConn1 -- BUS 46/RConn3 -- 2 39.2 kW 11 kV/LConn3
  Load Flow Bus43/LConn1 -- 2 6 kW 11 kV/LConn3 -- BUS 44/RConn3 -- Line 44-45/LConn3
  Line 53-54/LConn2 -- 43.5 kW 11 kV/LConn2 -- BUS 53/RConn2
  Load Flow Bus29/LConn1 -- BUS 30/RConn3 -- Line 30-31/LConn3
  100 kW 11 kV/LConn2 -- BUS 59/RConn2 -- Line 59-60/LConn2
  Line 56-57/LConn3 -- Load Flow Bus55/LConn1 -- BUS 56/RConn3
  Line 62-63/LConn2 -- 32 kW 11 kV/LConn2 -- BUS 62/RConn2
  1.2 kW 11 kV/LConn2 -- BUS 41/RConn2 -- Line 41-42/LConn2
  BUS 18/RConn1 -- 2 60 kW 11 kV/LConn1 -- Line 18-19/LConn1
  Load Flow Bus42/LConn1 -- 6 kW 11 kV/LConn3 -- Line 43-44/LConn3 -- BUS 43/RConn3
  BUS 25/RConn3 -- Load Flow Bus24/LConn1 -- Line 25-26/LConn3
  Load Flow Bus1/LConn1 -- Line 2-3/LConn3 -- BUS 2/RConn3
  2 28 kW 11 kV/LConn3 -- BUS 68/RConn3 -- Line 68-69/LConn3 -- Load Flow Bus67/LConn1
  Load Flow Bus6/LConn1 -- BUS 7/RConn3 -- Line 7-8/LConn3 -- 40 kW 11 kV/LConn3
  Line 51-52/LConn1 -- BUS 51/RConn1 -- 40.5 kW 11 kV/LConn1
  79 kW 11 kV/LConn3 -- BUS 48/RConn3 -- Line 48-49/LConn3 -- Load Flow Bus47/LConn1
  BUS 66/RConn2 -- 18 kW 11 kV/LConn2 -- Line 66-67/LConn2
  BUS 9/LConn3 -- 75 kW 11 kV/LConn3 -- Line 8-9/RConn3
  Load Flow Bus40/LConn1 -- 1.2 kW 11 kV/LConn3 -- Line 41-42/LConn3 -- BUS 41/RConn3
  Load Flow Bus17/LConn1 -- BUS 18/RConn3 -- Line 18-19/LConn3 -- 2 60 kW 11 kV/LConn3
  2 MW 11 kV/LConn3 -- Line 3-4/RConn3 -- BUS 4/LConn3
  BUS 14/RConn1 -- 2 8 kW 11 kV/LConn1 -- Line 14-15/LConn1
  Line 44-45/LConn1 -- 2 6 kW 11 kV/LConn1 -- BUS 44/RConn1
  Load Flow Bus56/LConn1 -- Line 57-58/LConn3 -- BUS 57/RConn3
  30 kW 11 kV/LConn1 -- Line 10-11/LConn1 -- BUS 10/RConn1
  Load Flow Bus20/LConn1 -- 114 kW 11 kV/LConn3 -- Line 21-22/LConn3 -- BUS 21/RConn3
  60 kW 11 kV/LConn3 -- BUS 17/RConn3 -- Line 17-18/LConn3 -- Load Flow Bus16/LConn1
  Load Flow Bus52/LConn1 -- 43.5 kW 11 kV/LConn3 -- Line 53-54/LConn3 -- BUS 53/RConn3
  Load Flow Bus3/LConn1 -- BUS 4/RConn3 -- Line 4-5/LConn3
  4 MW 11 kV/LConn2 -- 14 kW 11 kV/LConn2 -- Line 26-27/LConn2 -- BUS 26/RConn2
  2 MW 11 kV/LConn1 -- Line 3-4/RConn1 -- BUS 4/LConn1
  24 kW 11 kV/LConn1 -- BUS 39/RConn1 -- Line 39-40/LConn1
  30 kW 11 kV/LConn2 -- Line 10-11/LConn2 -- BUS 10/RConn2
  30 kW 11 kV/LConn1 -- Line 9-53/LConn1 -- BUS 9/RConn1 -- Line 9-10/LConn1
  Line 33-34/RConn1 -- BUS 34/LConn1
  Line 10-11/RConn2 -- BUS 11/LConn2
  Line 57-58/LConn1 -- BUS 57/RConn1
  BUS 11/LConn3 -- Line 10-11/RConn3
  BUS 41/LConn2 -- Line 40-41/RConn2
  Line 45-46/RConn3 -- BUS 46/LConn3
  Line 58-59/RConn1 -- BUS 59/LConn1
  BUS 16/LConn1 -- Line 15-16/RConn1
  Line 9-53/RConn3 -- BUS 53/LConn3
  Line 58-59/RConn2 -- BUS 59/LConn2
  3 28 kW 11 kV/LConn2 -- BUS 69/RConn2
  Line 22-23/RConn2 -- BUS 23/LConn2
  BUS 54/LConn2 -- Line 53-54/RConn2
  Line 62-63/RConn3 -- BUS 63/LConn3
  Line 19-20/LConn1 -- BUS 19/RConn1
  Line 12-68/RConn3 -- BUS 68/LConn3
  Line 29-30/RConn1 -- BUS 30/LConn1
  Line 1-2/RConn1 -- BUS 2/LConn1
  BUS 16/LConn3 -- Line 15-16/RConn3
  3.6 kW 11 kV/LConn1 -- BUS 52/RConn1
  Line 47-48/RConn1 -- BUS 48/LConn1
  Line 19-20/RConn1 -- BUS 20/LConn1
  Line 57-58/LConn2 -- BUS 57/RConn2
  Line 4-47/RConn1 -- BUS 47/LConn1
  Line 57-58/RConn3 -- BUS 58/LConn3
  Line 68-69/RConn3 -- BUS 69/LConn3
  Line 7-8/RConn1 -- BUS 8/LConn1
  BUS 37/LConn2 -- Line 36-37/RConn2
  Line 12-13/RConn3 -- BUS 13/LConn3
  BUS 10/LConn1 -- Line 9-10/RConn1
  Line 63-64/LConn2 -- BUS 63/RConn2
  BUS 7/LConn3 -- Line 6-7/RConn3
  BUS 27/LConn2 -- Line 26-27/RConn2
  Line 2-3/RConn1 -- BUS 3/LConn1
  Line 12-13/RConn1 -- BUS 13/LConn1
  Line 31-32/RConn1 -- BUS 32/LConn1
  Line 64-65/RConn2 -- BUS 65/LConn2
  Three-Phase Parallel RLC Load23/LConn2 -- BUS 27/RConn2
  Line 26-27/RConn1 -- BUS 27/LConn1
  BUS 51/LConn3 -- Line 8-51/RConn3
  Line 25-26/LConn2 -- BUS 25/RConn2
  Line 5-6/LConn2 -- BUS 5/RConn2
  2 18 kW 11 kV/LConn2 -- BUS 67/RConn2
  Line 18-19/RConn1 -- BUS 19/LConn1
  Line 60-61/RConn3 -- BUS 61/LConn3
  Line 47-48/RConn2 -- BUS 48/LConn2
  Line 12-68/RConn1 -- BUS 68/LConn1
  BUS 51/LConn2 -- Line 8-51/RConn2
  BUS 44/LConn2 -- Line 43-44/RConn2
  Line 26-27/RConn3 -- BUS 27/LConn3
  BUS 1/LConn1 -- G 1 11 kV Swing/RConn1
  BUS 56/RConn1 -- Line 56-57/LConn1
  BUS 38/LConn2 -- Line 37-38/RConn2
  Line 36-37/LConn1 -- BUS 36/RConn1
  Line 36-37/RConn3 -- BUS 37/LConn3
  Line 44-45/RConn3 -- BUS 45/LConn3
  BUS 24/LConn2 -- Line 23-24/RConn2
  Line 56-57/RConn1 -- BUS 57/LConn1
  Line 32-33/LConn2 -- BUS 32/RConn2
  Line 5-6/LConn1 -- BUS 5/RConn1
  Line 1-2/RConn3 -- BUS 2/LConn3
  Line 59-60/RConn1 -- BUS 60/LConn1
  Line 36-37/RConn1 -- BUS 37/LConn1
  Line 25-26/RConn1 -- BUS 26/LConn1
  Line 7-8/RConn3 -- BUS 8/LConn3
  BUS 6/LConn1 -- Line 5-6/RConn1
  BUS 10/LConn3 -- Line 9-10/RConn3
  BUS 42/LConn2 -- Line 41-42/RConn2
  BUS 45/LConn2 -- Line 44-45/RConn2
  BUS 25/LConn2 -- Line 24-25/RConn2
  Line 12-68/RConn2 -- BUS 68/LConn2
  Line 48-49/RConn3 -- BUS 49/LConn3
  Line 22-23/RConn1 -- BUS 23/LConn1
  Line 40-41/RConn1 -- BUS 41/LConn1
  Line 63-64/RConn1 -- BUS 64/LConn1
  Line 43-44/RConn3 -- BUS 44/LConn3
  Line 58-59/LConn2 -- BUS 58/RConn2
  Line 3-28/RConn1 -- BUS 28/LConn1
  Line 19-20/RConn3 -- BUS 20/LConn3
  Line 38-39/RConn1 -- BUS 39/LConn1
  BUS 1/LConn3 -- G 1 11 kV Swing/RConn3
  Line 38-39/LConn2 -- BUS 38/RConn2
  Line 55-56/LConn2 -- BUS 55/RConn2
  Line 20-21/RConn3 -- BUS 21/LConn3
  BUS 17/LConn2 -- Line 16-17/RConn2
  Line 38-39/LConn1 -- BUS 38/RConn1
  Line 44-45/RConn1 -- BUS 45/LConn1
  Line 30-31/RConn1 -- BUS 31/LConn1
  Line 60-61/RConn1 -- BUS 61/LConn1
  Line 60-61/RConn2 -- BUS 61/LConn2
  BUS 15/LConn1 -- Line 14-15/RConn1
  Line 19-20/LConn2 -- BUS 19/RConn2
  BUS 60/LConn2 -- Line 59-60/RConn2
  2 39.2 kW 11 kV/LConn2 -- BUS 46/RConn2
  Line 62-63/RConn1 -- BUS 63/LConn1
  Line 55-56/RConn1 -- BUS 56/LConn1
  BUS 49/LConn2 -- Line 48-49/RConn2
  Line 60-61/LConn2 -- BUS 60/RConn2
  Line 13-14/RConn1 -- BUS 14/LConn1
  BUS 26/LConn2 -- Line 25-26/RConn2
  Line 53-54/RConn1 -- BUS 54/LConn1
  BUS 20/LConn2 -- Line 19-20/RConn2
  Line 39-40/RConn2 -- BUS 40/LConn2
  Line 37-38/RConn1 -- BUS 38/LConn1
  Line 51-52/RConn1 -- BUS 52/LConn1
  Three-Phase Parallel RLC Load23/LConn1 -- BUS 27/RConn1
  59 kW 11 kV/LConn1 -- BUS 65/RConn1
  Line 4-5/LConn2 -- BUS 4/RConn2
  Line 2-3/RConn3 -- BUS 3/LConn3
  Line 49-50/RConn1 -- BUS 50/LConn1
  Line 57-58/RConn2 -- BUS 58/LConn2
  Line 54-55/RConn3 -- BUS 55/LConn3
  59 kW 11 kV/LConn2 -- BUS 65/RConn2
  Line 28-29/RConn3 -- BUS 29/LConn3
  Line 55-56/RConn3 -- BUS 56/LConn3
  Line 57-58/RConn1 -- BUS 58/LConn1
  Line 68-69/RConn1 -- BUS 69/LConn1
  Line 59-60/RConn3 -- BUS 60/LConn3
  BUS 19/LConn2 -- Line 18-19/RConn2
  2 384.7 kW 11 kV/LConn1 -- BUS 50/RConn1
  Line 10-11/RConn1 -- BUS 11/LConn1
  Line 2-3/RConn2 -- BUS 3/LConn2
  2 39.2 kW 11 kV/LConn1 -- BUS 46/RConn1
  Line 42-43/RConn1 -- BUS 43/LConn1
  Line 66-67/RConn3 -- BUS 67/LConn3
  Line 24-25/LConn1 -- BUS 24/RConn1
  Line 24-25/LConn2 -- BUS 24/RConn2
  Line 17-18/RConn1 -- BUS 18/LConn1
  BUS 39/LConn2 -- Line 38-39/RConn2
  Line 49-50/RConn3 -- BUS 50/LConn3
  Line 4-47/RConn2 -- BUS 47/LConn2
  BUS 31/RConn1 -- Line 31-32/LConn1
  Line 47-48/RConn3 -- BUS 48/LConn3
  Line 24-25/RConn1 -- BUS 25/LConn1
  Line 20-21/RConn1 -- BUS 21/LConn1
  Line 15-16/LConn1 -- BUS 15/RConn1
  BUS 12/LConn3 -- Line 11-12/RConn3
  Line 1-2/LConn2 -- BUS 1/RConn2
  Line 63-64/RConn3 -- BUS 64/LConn3
  Line 3-28/RConn3 -- BUS 28/LConn3
  Line 53-54/RConn3 -- BUS 54/LConn3
  Line 32-33/RConn1 -- BUS 33/LConn1
  2 18 kW 11 kV/LConn1 -- BUS 67/RConn1
  BUS 25/RConn1 -- Line 25-26/LConn1
  Line 33-34/RConn2 -- BUS 34/LConn2
  Line 42-43/LConn2 -- BUS 42/RConn2
  Line 56-57/LConn2 -- BUS 56/RConn2
  Line 61-62/RConn3 -- BUS 62/LConn3
  Line 55-56/RConn2 -- BUS 56/LConn2
  BUS 22/LConn2 -- Line 21-22/RConn2
  BUS 13/LConn2 -- Line 12-13/RConn2
  3 28 kW 11 kV/LConn1 -- BUS 69/RConn1
  BUS 15/LConn3 -- Line 14-15/RConn3
  BUS 7/LConn2 -- Line 6-7/RConn2
  Line 47-48/LConn1 -- BUS 47/RConn1
  Line 32-33/RConn3 -- BUS 33/LConn3
  Line 56-57/RConn2 -- BUS 57/LConn2
  BUS 21/LConn2 -- Line 20-21/RConn2
  BUS 12/LConn1 -- Line 11-12/RConn1
  Line 2-3/LConn2 -- BUS 2/RConn2
  BUS 18/LConn2 -- Line 17-18/RConn2
  Line 32-33/LConn1 -- BUS 32/RConn1
  Line 41-42/RConn3 -- BUS 42/LConn3
  Line 37-38/RConn3 -- BUS 38/LConn3
  Line 21-22/RConn3 -- BUS 22/LConn3
  BUS 15/LConn2 -- Line 14-15/RConn2
  Line 9-53/RConn1 -- BUS 53/LConn1
  3.6 kW 11 kV/LConn2 -- BUS 52/RConn2
  Three-Phase Parallel RLC Load42/LConn1 -- BUS 35/RConn1
  Line 63-64/RConn2 -- BUS 64/LConn2
  Line 43-44/RConn1 -- BUS 44/LConn1
  Line 30-31/RConn3 -- BUS 31/LConn3
  Line 39-40/RConn3 -- BUS 40/LConn3
  Line 5-6/RConn3 -- BUS 6/LConn3
  Line 49-50/RConn2 -- BUS 50/LConn2
  Line 5-6/RConn2 -- BUS 6/LConn2
  Line 13-14/RConn3 -- BUS 14/LConn3
  BUS 30/LConn2 -- Line 29-30/RConn2
  Line 42-43/RConn3 -- BUS 43/LConn3
  Line 4-5/LConn1 -- BUS 4/RConn1
  Line 3-28/RConn2 -- BUS 28/LConn2
  Line 29-30/RConn3 -- BUS 30/LConn3
  Line 64-65/RConn1 -- BUS 65/LConn1
  Line 36-37/LConn2 -- BUS 36/RConn2
  BUS 31/LConn2 -- Line 30-31/RConn2
  BUS 66/LConn2 -- Line 11-66/RConn2
  Line 60-61/LConn1 -- BUS 60/RConn1
  Line 51-52/RConn2 -- BUS 52/LConn2
  Line 17-18/RConn3 -- BUS 18/LConn3
  BUS 66/LConn3 -- Line 11-66/RConn3
  Three-Phase Parallel RLC Load42/LConn2 -- BUS 35/RConn2
  Line 31-32/LConn2 -- BUS 31/RConn2
  Line 41-42/RConn1 -- BUS 42/LConn1
  Line 16-17/LConn1 -- BUS 16/RConn1
  Line 1-2/RConn2 -- BUS 2/LConn2
  Line 30-31/LConn2 -- BUS 30/RConn2
  Line 28-29/RConn1 -- BUS 29/LConn1
  Line 25-26/RConn3 -- BUS 26/LConn3
  Line 34-35/RConn1 -- BUS 35/LConn1
  Line 18-19/RConn3 -- BUS 19/LConn3
  Line 6-7/LConn2 -- BUS 6/RConn2
  BUS 32/LConn2 -- Line 31-32/RConn2
  Line 6-7/LConn1 -- BUS 6/RConn1
  Line 21-22/RConn1 -- BUS 22/LConn1
  Line 1-2/LConn1 -- BUS 1/RConn1
  BUS 10/LConn2 -- Line 9-10/RConn2
  Line 45-46/RConn1 -- BUS 46/LConn1
  Line 34-35/RConn2 -- BUS 35/LConn2
  BUS 12/LConn2 -- Line 11-12/RConn2
  Line 63-64/LConn1 -- BUS 63/RConn1
  BUS 1/LConn2 -- G 1 11 kV Swing/RConn2
  BUS 43/LConn2 -- Line 42-43/RConn2
  Line 48-49/RConn1 -- BUS 49/LConn1
  Line 33-34/RConn3 -- BUS 34/LConn3
  Line 54-55/RConn1 -- BUS 55/LConn1
  Line 55-56/LConn1 -- BUS 55/RConn1
  Line 34-35/RConn3 -- BUS 35/LConn3
  Line 39-40/RConn1 -- BUS 40/LConn1
  Line 40-41/RConn3 -- BUS 41/LConn3
  Line 38-39/RConn3 -- BUS 39/LConn3
  BUS 29/LConn2 -- Line 28-29/RConn2
  BUS 42/RConn1 -- Line 42-43/LConn1
  BUS 46/LConn2 -- Line 45-46/RConn2
  2 384.7 kW 11 kV/LConn2 -- BUS 50/RConn2
  Line 51-52/RConn3 -- BUS 52/LConn3
  BUS 66/LConn1 -- Line 11-66/RConn1
  Line 23-24/RConn3 -- BUS 24/LConn3
  Line 15-16/LConn2 -- BUS 15/RConn2
  BUS 16/LConn2 -- Line 15-16/RConn2
  Line 47-48/LConn2 -- BUS 47/RConn2
  Line 16-17/RConn1 -- BUS 17/LConn1
  Line 23-24/RConn1 -- BUS 24/LConn1
  BUS 14/LConn2 -- Line 13-14/RConn2
  Line 61-62/RConn2 -- BUS 62/LConn2
  BUS 33/LConn2 -- Line 32-33/RConn2
  Line 61-62/RConn1 -- BUS 62/LConn1
  Line 66-67/RConn2 -- BUS 67/LConn2
  Line 22-23/RConn3 -- BUS 23/LConn3
  Line 62-63/RConn2 -- BUS 63/LConn2
  Line 68-69/RConn2 -- BUS 69/LConn2
  BUS 55/LConn2 -- Line 54-55/RConn2
  Line 64-65/RConn3 -- BUS 65/LConn3
  Line 16-17/LConn2 -- BUS 16/RConn2
  Line 66-67/RConn1 -- BUS 67/LConn1
  Line 2-3/LConn1 -- BUS 2/RConn1
  Line 24-25/RConn3 -- BUS 25/LConn3
  BUS 51/LConn1 -- Line 8-51/RConn1
  BUS 7/LConn1 -- Line 6-7/RConn1
  Line 16-17/RConn3 -- BUS 17/LConn3
  Line 4-47/RConn3 -- BUS 47/LConn3
  Line 58-59/RConn3 -- BUS 59/LConn3
  Line 9-53/RConn2 -- BUS 53/LConn2
  Line 58-59/LConn1 -- BUS 58/RConn1
  Line 31-32/RConn3 -- BUS 32/LConn3
  Line 30-31/LConn1 -- BUS 30/RConn1
  Line 56-57/RConn3 -- BUS 57/LConn3
  Line 7-8/RConn2 -- BUS 8/LConn2
